simulink library "etherlab_lib"  (Simulink 7.4)
settings: Solver=ode45  SolverMode=SingleTasking  StartTime=0.0  StopTime=10.0  RelTol=1e-3
undefined symbols (not defined in the file or in its folder): Address, baumer_ecatencoder, el320x, el500x, el5101, el5101_0010, EL5151, El5152, el515x, ep41xx, ep43xx, rv, x
(part 2 of 3)

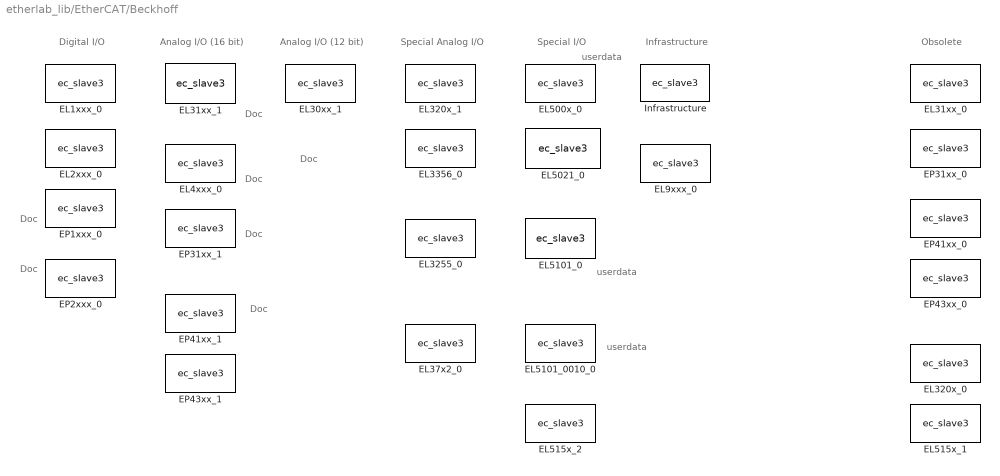
== system etherlab_lib/EtherCAT/Beckhoff ==
  note: Analog I/O (16 bit)
  note: Digital I/O
  note: Analog I/O (12 bit)
  note: Special Analog I/O
  note: Special I/O
  note: Infrastructure
  note: Obsolete
  note: Doc
  note: Doc
  note: Doc
  note: Doc
  note: Doc
  note: Doc
  note: Doc
  note: userdata
  note: userdata
  note: userdata
  EL1xxx_0 : S-Function  FunctionName=ec_slave3  Parameters=Address,rv.SlaveConfig,rv.PortConfig,debug,tsample  SFunctionModules='ecrt_support'  EnableBusSupport=off  mask(EL1xxx){master=0, index=1, model=EL1004, vector=on, tsample=0, debug=0}
      mask prompts: index "Slave Index"; model "Device Model"; vector "Vector Outputs"; tsample "Sample Time"; debug "Debug Level"
      mask help: Beckhoff EtherCAT Digital Input
      mask init:
      | Address = getEtherCATAddress(gcb, master, index, tsample);
      | 
      | rv = el1xxx.configure(model,vector);
      mask Help: web(etherlab_help_path('el1xxx.html'), '-helpbrowser');
      mask StyleString: edit,edit,popup(EL1002|EL1004|EL1004-0010|EL1008|EL1012|EL1014|EL1018|EL1024|EL1034|EL1084|EL1088|EL1094|EL1098|EL1104|EL1114|EL1124|EL1134|EL1144|EL1202|EL1702|EL1712|EL1722|EL1804|EL1808|EL1809|EL1814|EL1819|EL1862|EL1872|EL1889|EL1014-0000-0000),checkbox,edit,edit
      mask Display: fprintf('%s\nM:%i Idx:%s', model, master, mat2str(index))
  EL2xxx_0 : S-Function  FunctionName=ec_slave3  Parameters=Address,rv.SlaveConfig,rv.PortConfig,debug,tsample  SFunctionModules='ecrt_support'  EnableBusSupport=off  mask(EL2xxx){master=0, index=1, model=EL2004, vector=on, diag=on, tsample=-1, debug=0}
      mask prompts: index "Slave Index"; model "Device Model"; vector "Vector Inputs"; diag "Diag Port"; tsample "Sample Time (-1 for inherited)"
      mask help: Beckhoff EtherCAT Digital Output
      mask init:
      | Address = getEtherCATAddress(gcb, master, index, tsample);
      | 
      | rv = el2xxx.configure(model,vector,diag);
      mask Help: web(etherlab_help_path('el2xxx.html'), '-helpbrowser')
      mask StyleString: edit,edit,popup(EL2002|EL2004|EL2008|EL2022|EL2024|EL2032|EL2034|EL2042|EL2084|EL2088|EL2124|EL2202|EL2602|EL2612|EL2622|EL2624|EL2712|EL2722|EL2732|EL2798|EL2808|EL2809|EL2004-0000-0000|EL2032-0000-0000),checkbox,checkbox,edit,edit
      mask CallbackString: ||EtherCATSlaveBlock().setEnable('diag',el2xxx.hasDiag(get_param(gcb,'model')))||||
      mask Display: fprintf('%s\nM:%i Idx:%s', model, master, mat2str(index))
  EL30xx_1 : S-Function  FunctionName=ec_slave3  Parameters=Address,rv.SlaveConfig,rv.PortConfig,debug,tsample  SFunctionModules='ecrt_support'  EnableBusSupport=off  mask(EL30xx){master=0, index=1, model=EL3002, vector=on, status=on, gain=, offset=, tau=, tsample=0, debug=0, filter=Off, opmode=FreeRun, fastop=off}
      mask prompts: index "Slave Index"; model "Device Model"; vector "Vector Output"; status "Status Output"; gain "Output Scale"; offset "Output Offset"; tau "LPF Time Constant (sec)"; tsample "Sample Time"; opmode "Synchronization Mode (1C33:01.0)"; fastop "FastOp Mode (1C33:01.15)"
      mask help: Beckhoff 1,2,4,8-Channel 16-Bit Analog Input
      mask init:
      | Address = getEtherCATAddress(gcb, master, index, tsample);
      | 
      | rv = el30xx_1.configure(model,status,vector,...
      |     EtherCATSlave.configureScale(2^15,gain,offset,tau),...
      |     [filter,opmode,fastop]);
      | 
      | EtherCATSlaveBlock().setPortNames({},...
      |     {rv.PortConfig.output.portname})
      | 
      | set_param(gcb,'AttributesFormatString',...
      |     sprintf('%s %s\nM:%i Idx:%s',...
      |             model,rv.function,master,mat2str(index)))
      settings: AttributesFormatString=|
      | EL3002 +-10V
      | M:0 Idx:1
      mask StyleString: edit,edit,popup(EL3001|EL3002|EL3004|EL3008|EL3011|EL3012|EL3014|EL3021|EL3022|EL3024|EL3041|EL3042|EL3044|EL3048|EL3051|EL3052|EL3054|EL3058|EL3061|EL3062|EL3062-0030|EL3064|EL3068),checkbox,checkbox,edit,edit,edit,edit,edit,popup(Off|50Hz FIR|60Hz FIR|IIR 1|IIR 2|IIR 3|IIR 4|IIR 5|IIR 6|IIR 7|IIR 8),popup(FreeRun|FrameTriggered SM2),checkbox
      mask CallbackString:
      | ||||||||||EtherCATSlaveBlock().setEnable({'opmode','fastop'},...
      |         strcmp(get_param(gcb,'filter'),'Off'));
      | ||
      mask TabNameString: Main,Main,Main,Main,Main,Main,Main,Main,Main,Main,Filter,Filter,Filter
      mask Display:
      | port_label('output', 1, 'Value')
      | port_label('output', 2, 'Status')
  EL31xx_0 : S-Function  LoadFcn=|  FunctionName=ec_slave3  Parameters=Address,rv.SlaveConfig,rv.PortConfig,debug,tsample  SFunctionModules='ecrt_support'  EnableBusSupport=off  mask(EL31xx){master=0, index=1, model=EL3102, dc=DC-Synchron, vector=on, raw=off, scale=, offset=, tau=, tsample=0, debug=0}
      | el31xx('check')                              
      | if ~strcmp(bdroot(gcb),'etherlab_lib')       
      |    disp([gcb ' is obsolete. Please replace'])
      | end
      mask prompts: index "Slave Index"; model "Device Model"; dc "Distributed Clock"; vector "Vector Output"; raw "Raw output"; scale "Output Scale"; offset "Output Offset"; tau "LPF Time Constant (sec)"; tsample "Sample Time"
      mask help:
      | Beckhoff 2,4,8-Channel 16-Bit Analog Input with Distributed Clocks
      |
      | Status output is not supported
      mask init:
      | masterStr = '';
      | positionStr = '';
      | [Address masterStr positionStr] = ...
      |     getEtherCATAddress(gcb, master, index, tsample);
      | 
      | el31xx('set');  % Report errors
      | 
      | rv = get_param(gcb,'UserData');
      mask Help:
      | This block generically implements the EtherCAT 16-Bit Analog Input Terminal for various models.
      | <p/>
      | The following Terminals are supported:
      | <center>
      | <table width="80%">
      | <tr><td>EL3102,4,8</td><td>-10..10V Voltage Input</td></tr>
      | <tr><td>EL3112,4   </td><td>0..20mA Current Input</td></tr>
      | <tr><td>EL3122,4   </td><td>4..20mA Current Input</td></tr>
      | <tr><td>EL3142,4,8</td><td>0..20mA Current Input</td></tr>
      | <tr><td>EL3152,4,8</td><td>4..20mA Current Input</td></tr>
      | <tr><td>EL3162,4,8</td><td>0..10V Voltage Input</td></tr>
      | </table>
      | </center>
      | <p/>
      | Choose and set the following options:
      | <h4>Master:</h4>
      | Set the EtherCAT Master of this terminal.
      | 
      | <h4>Slave Index:</h4>
      | Set the EtherCAT slave index. Following address formats are allowed:
      | <ol>
      | <li> Absolute addressing: a scalar number <<b><tt>n</tt></b>> representing the (zero based) absolute position in the bus.
      | <li> SSId addressing: the Secondary Slave (or 'Alias') Addressing has the form <<b><tt>[alias position]</tt></b>> where <b><tt>alias</tt></b> is the Secondary Slave Id of the EtherCAT slave and <b><tt>position</tt></b> is the offset after the slave with the given <b><tt>alias</tt></b>. The SSId has to be preprogrammed into the slave with other service tools (see 'ethercat alias --help').
      | </ol>
      | 
      | <h4>Device Model:</h4>
      | Choose the model at the Indexed position of the master.
      | 
      | <h4>Output Type:</h4>
      | <ul>
      | <li>Choose <b>Vector Output</b> to have a single output as a vector
      | with a size corresponding to the channel count of the terminal. This mode also allows a status output port to be displayed. <br/>
      | <li>Choose <b>Separate Outputs</b> to have one output for every channel.
      | </ul>
      | <h4>Output Full Scale</h4>
      | When <b>Output Data Type</b> is set to <b>Double with scale and offset</b>, the block's output value at full scale terminal input can be set here.
      | 
      | <h4>Output Offset</h4>
      | When <b>Output Data Type</b> is set to <b>Double with scale and offset</b>, the blocks output at zero terminal input can be set here. Note that the Full Scale above is also increased by this amount. Note furthermore that this corresponds to the minimum input for terminals such as 4..20mA.
      | 
      | <h4>Output Data Type</h4>
      | Choose the block's output data type for the output signal. Available are:
      | <ul>
      | <li><b><tt>Raw</tt></b> outputting the internal raw value as <tt>int16_T</tt> or <tt>uint16_T</tt> as appropriate
      | <li><b><tt>Double</tt></b> outputting 0..10, -10..10, 0..0.02 and 0.004..0.02 depending on the Model as appropriate
      | <li><b><tt>Double with scale and offset</tt></b>, allowing the output to be scaled with an offset.
      | </ul>
      | 
      | <p>
      | Choosing <b>Status Output</b> provides a port of type <tt>uint8_T</tt> where the status is presented. This is only enabled when <b>Vector Output</b> is selected. Terminal input over- and underrange can be detected using this output. See the terminal's documentation.
      | 
      | <h4>Output Filter</h4>
      | When not in <b>Raw</b> mode, the <b>Output Filter</b> checkbox becomes available, allowing the use of an internal low pass filter. Enter the <b>LPF Time Constant</b> for the filter in the field below.
      | <br>For continuous sample time systems (0 in Sample Time), the filter is also continuous. Discrete samples systems (Sample Time > 0) uses an equivalent discrete low pass filter with a similar time constant.
      | 
      | <p>
      | Set the <b>Sample Time</b> for the block. <tt>0</tt> is continuous sample time (runs at the model's base rate). Setting <tt>-1</tt> will try to set the time using back propagation.
      mask StyleString: edit,edit,popup(EL3101|EL3102|EL3104|EL3111|EL3112|EL3114|EL3121|EL3122|EL3124|EL3141|EL3142|EL3142-010|EL3144|EL3151|EL3152|EL3154|EL3161|EL3162|EL3164),popup(Free Run|DC-Synchron|DC-Synchron (input based)),checkbox,checkbox,edit,edit,edit,edit,edit
      mask CallbackString: ||el31xx('set')|el31xx('set')|el31xx('set')||||||
      mask Display:
      | fprintf('%s\n%s AIn\nM:%s Idx:%s', ...
      |     model, rv.SlaveConfig.function, masterStr, positionStr)
  EL31xx_1 : S-Function  FunctionName=ec_slave3  Parameters=Address,rv.SlaveConfig,rv.PortConfig,debug,tsample  SFunctionModules='ecrt_support'  EnableBusSupport=off  mask(EL31xx){master=0, index=1, model=EL3102, vector=on, status=on, filter=Off, gain=, offset=, tau=, tsample=0, debug=, dc_mode=Free Run/SM-Synchron, dc_assign_activate=, dc_cycle0=[], dc_cycle0_factor=[], dc_shift0=[], dc_shift0_factor=[], dc_shift0_input=off, dc_cycle1=[], dc_cycle1_factor=[], dc_shift1=[], dc_shift1_factor=[]}
      mask prompts: index "Slave Index"; model "Device Model"; vector "Vector Output"; status "Status output"; gain "Output Gain"; offset "Output Offset"; tau "LPF Time Constant (sec)"; tsample "Sample Time"; dc_mode "Mode"; dc_assign_activate "Assign Activate"; dc_cycle0 "Cycle Time Sync 0"; dc_cycle0_factor "Factor"; dc_shift0 "Shift Time Sync0"; dc_shift0_factor "Factor"; dc_shift0_input "Shift Time0 Input"; dc_cycle1 "Cycle Time Sync1"; dc_cycle1_factor "Factor"; dc_shift1 "Shift Time Sync1"; dc_shift1_factor "Factor"
      mask help: Beckhoff 2,4,8-Channel 16-Bit Analog Input with Distributed Clocks
      mask init:
      | Address = getEtherCATAddress(gcb, master, index, tsample);
      | 
      | rv = el31xx_1.configure(model,status,vector,...
      |     EtherCATSlave.configureScale(2^15,gain,offset,tau),...
      |     [dc_mode, dc_assign_activate, ...
      |      dc_cycle0, dc_cycle0_factor, ...
      |      dc_shift0, dc_shift0_factor, dc_shift0_input, ...
      |      dc_cycle1, dc_cycle1_factor, ...
      |      dc_shift1, dc_shift1_factor], ...
      |      filter);
      |  
      | EtherCATSlaveBlock().setPortNames({},...
      |     {rv.PortConfig.output.portname})
      | 
      | set_param(gcb,'AttributesFormatString',...
      |     sprintf('%s %s\nM:%i Idx:%s',...
      |             model,rv.function,master,mat2str(index)))
      settings: AttributesFormatString=|
      | EL3102 +-10V
      | M:0 Idx:1
      mask Help:
      | This block generically implements the EtherCAT 16-Bit Analog Input Terminal for various models.
      | <p/>
      | The following Terminals are supported:
      | <center>
      | <table width="80%">
      | <tr><td>EL3102,4,8</td><td>-10..10V Voltage Input</td></tr>
      | <tr><td>EL3112,4   </td><td>0..20mA Current Input</td></tr>
      | <tr><td>EL3122,4   </td><td>4..20mA Current Input</td></tr>
      | <tr><td>EL3142,4,8</td><td>0..20mA Current Input</td></tr>
      | <tr><td>EL3152,4,8</td><td>4..20mA Current Input</td></tr>
      | <tr><td>EL3162,4,8</td><td>0..10V Voltage Input</td></tr>
      | </table>
      | </center>
      | <p/>
      | Choose and set the following options:
      | <h4>Master:</h4>
      | Set the EtherCAT Master of this terminal.
      | 
      | <h4>Slave Index:</h4>
      | Set the EtherCAT slave index. Following address formats are allowed:
      | <ol>
      | <li> Absolute addressing: a scalar number <<b><tt>n</tt></b>> representing the (zero based) absolute position in the bus.
      | <li> SSId addressing: the Secondary Slave (or 'Alias') Addressing has the form <<b><tt>[alias position]</tt></b>> where <b><tt>alias</tt></b> is the Secondary Slave Id of the EtherCAT slave and <b><tt>position</tt></b> is the offset after the slave with the given <b><tt>alias</tt></b>. The SSId has to be preprogrammed into the slave with other service tools (see 'ethercat alias --help').
      | </ol>
      | 
      | <h4>Device Model:</h4>
      | Choose the model at the Indexed position of the master.
      | 
      | <h4>Output Type:</h4>
      | <ul>
      | <li>Choose <b>Vector Output</b> to have a single output as a vector
      | with a size corresponding to the channel count of the terminal. This mode also allows a status output port to be displayed. <br/>
      | <li>Choose <b>Separate Outputs</b> to have one output for every channel.
      | </ul>
      | <h4>Output Full Scale</h4>
      | When <b>Output Data Type</b> is set to <b>Double with scale and offset</b>, the block's output value at full scale terminal input can be set here.
      | 
      | <h4>Output Offset</h4>
      | When <b>Output Data Type</b> is set to <b>Double with scale and offset</b>, the blocks output at zero terminal input can be set here. Note that the Full Scale above is also increased by this amount. Note furthermore that this corresponds to the minimum input for terminals such as 4..20mA.
      | 
      | <h4>Output Data Type</h4>
      | Choose the block's output data type for the output signal. Available are:
      | <ul>
      | <li><b><tt>Raw</tt></b> outputting the internal raw value as <tt>int16_T</tt> or <tt>uint16_T</tt> as appropriate
      | <li><b><tt>Double</tt></b> outputting 0..10, -10..10, 0..0.02 and 0.004..0.02 depending on the Model as appropriate
      | <li><b><tt>Double with scale and offset</tt></b>, allowing the output to be scaled with an offset.
      | </ul>
      | 
      | <p>
      | Choosing <b>Status Output</b> provides a port of type <tt>uint8_T</tt> where the status is presented. This is only enabled when <b>Vector Output</b> is selected. Terminal input over- and underrange can be detected using this output. See the terminal's documentation.
      | 
      | <h4>Output Filter</h4>
      | When not in <b>Raw</b> mode, the <b>Output Filter</b> checkbox becomes available, allowing the use of an internal low pass filter. Enter the <b>LPF Time Constant</b> for the filter in the field below.
      | <br>For continuous sample time systems (0 in Sample Time), the filter is also continuous. Discrete samples systems (Sample Time > 0) uses an equivalent discrete low pass filter with a similar time constant.
      | 
      | <p>
      | Set the <b>Sample Time</b> for the block. <tt>0</tt> is continuous sample time (runs at the model's base rate). Setting <tt>-1</tt> will try to set the time using back propagation.
      mask StyleString: edit,edit,popup(EL3101|EL3102|EL3104|EL3111|EL3112|EL3114|EL3121|EL3122|EL3124|EL3141|EL3142|EL3142-0010|EL3144|EL3151|EL3152|EL3154|EL3161|EL3162|EL3164),checkbox,checkbox,popup(Off|50Hz FIR|60Hz FIR|IIR 1|IIR 2|IIR 3|IIR 4|IIR 5|IIR 6|IIR 7|IIR 8),edit,edit,edit,edit,edit,popup(Free Run/SM-Synchron|DC-Synchron|DC-Synchron (input based)|Custom),edit,min,max,min,max,checkbox,min,max,min,max
      mask CallbackString: |||||||||||EtherCATSlaveBlock().updateCustomDCEnable()||||||||||
      mask TabNameString: Main,Main,Main,Main,Main,Main,Main,Main,Main,Main,Main,Distributed Clocks,Distributed Clocks,Distributed Clocks,Distributed Clocks,Distributed Clocks,Distributed Clocks,Distributed Clocks,Distributed Clocks,Distributed Clocks,Distributed Clocks,Distributed Clocks
      mask Display:
      | port_label('output', 1, 'Value')
      | port_label('output', 2, 'Status')
  EL320x_0 : S-Function  LoadFcn=el320x('check')  FunctionName=ec_slave3  Parameters=Address,rv.SlaveConfig,rv.PortConfig,debug,tsample  SFunctionModules='ecrt_support'  EnableBusSupport=off  mask(EL320x){master=0, index=1, model=EL3204, rtd=0, technology=2, filter=50 Hz, vector=on, enable_status=on, tsample=0, debug=0}
      mask prompts: index "Slave Index"; model "Device Model"; rtd "RTD-Element (CoE 80x0:19)"; technology "Connection Technology (CoE 80x0:1A)"; filter "Filter (CoE 8000:15)"; vector "Vector Output"; enable_status "Status Port"; tsample "Sample Time"
      mask help: Beckhoff 1, 2, 4-Channel Input Terminal Pt100 (RTD)
      mask init:
      | masterStr = '';
      | positionStr = '';
      | [Address masterStr positionStr] = ...
      |     getEtherCATAddress(gcb,master,index,tsample);
      | SdoConfig = [];
      | 
      | rv = get_param(gcbh,'UserData');
      | 
      | count = numel(rv.SlaveConfig.sm{1}{3});
      | 
      | err = {};
      | if numel(rtd) == 1
      |     rtd = repmat(rtd,1,count);
      | elseif numel(rtd) ~= count
      |     err = {['- Mask option "RTD Element"' ...
      |         ' is not a scalar or vector with ' ...
      |         num2str(count) ' elements']};
      | end
      | 
      | if numel(technology) == 1
      |     technology = repmat(technology,1,count);
      | elseif numel(technology) ~= count
      |     err = horzcat(err, ['- Mask option "Connection Technology"' ...
      |         ' is not a scalar or vector with ' ...
      |         num2str(count) ' elements']);
      | end
      | 
      | if ~isempty(err)
      |     errordlg(err,gcb);
      |     return
      | end
      | 
      | rv.SlaveConfig.sdo = num2cell(vertcat(...
      |     [hex2dec('8000'),6,8,1],...
      |     [hex2dec('8000'),hex2dec('15'),16,filter+1],...
      |     horzcat(repmat(hex2dec('8000') + 16*(0:count-1)',2,1),...
      |             [hex2dec('19')*ones(count,1);hex2dec('1a')*ones(count,1)],...
      |             16*ones(count*2,1),...
      |             vertcat(reshape(rtd,[],1),...
      |                     reshape(technology,[],1)))));
      mask Help: web(etherlab_help_path('el320x.html'), '-helpbrowser');
      mask StyleString: edit,edit,popup(EL3201|EL3201-0010|EL3201-0020|EL3202|EL3202-0010|EL3204),edit,edit,popup(50 Hz|60 Hz|100 Hz|500 Hz|1 kHz|2 kHz|3.75 kHz|7.5 kHz|15 kHz|30 kHz|5 Hz|10 Hz),checkbox,checkbox,edit,edit
      mask CallbackString: ||el320x('set');||||el320x('set');|el320x('set');||
      mask Display: fprintf('%s\nRTD In\n%i Idx:%s', model, master, mat2str(index))
  EL320x_1 : S-Function  FunctionName=ec_slave3  Parameters=Address,rv.SlaveConfig,rv.PortConfig,debug,tsample  SFunctionModules='ecrt_support'  EnableBusSupport=off  mask(EL320x){master=0, index=1, model=EL3204, filter=Off, vector=on, status=on, tsample=0, debug=, rtd1=Pt100 -200...850C, technology1=2-wire, calib1=0, rtd2=Pt100 -200...850C, technology2=2-wire, calib2=0, rtd3=Pt100 -200...850C, technology3=2-wire, calib3=0, rtd4=Pt100 -200...850C, technology4=2-wire, calib4=0}
      mask prompts: index "Slave Index"; model "Device Model"; vector "Vector Output"; status "Status Port"; tsample "Sample Time"; rtd1 "RTD-Element"; technology1 "Technology"; calib1 "Wire Calibration (1/32 Ohm)"; rtd2 "RTD-Element"; technology2 "Technology"; calib2 "Wire Calibration (1/32 Ohm)"; rtd3 "RTD-Element"; technology3 "Technology"; calib3 "Wire Calibration (1/32 Ohm)"; rtd4 "RTD-Element"; technology4 "Technology"; calib4 "Wire Calibration (1/32 Ohm)"
      mask help: Beckhoff 1, 2, 4-Channel Input Terminal Pt100 (RTD)
      mask init:
      | Address = getEtherCATAddress(gcb,master,index,tsample);
      | 
      | % rv.SlaveConfig.sdo = num2cell(vertcat(...
      | %     [hex2dec('8000'),6,8,1],...
      | %     [hex2dec('8000'),hex2dec('15'),16,filter+1],...
      | %     horzcat(repmat(hex2dec('8000') + 16*(0:count-1)',2,1),...
      | %             [hex2dec('19')*ones(count,1);hex2dec('1a')*ones(count,1)],...
      | %             16*ones(count*2,1),...
      | %             vertcat(reshape(rtd,[],1),...
      | %                     reshape(technology,[],1)))));
      | % rv.PortConfig = [];
      | % rv.SlaveConfig = [];
      | 
      | rv = el320x_1.configure(model,status,vector,filter,...
      |     [rtd1,rtd2,rtd3,rtd4],...
      |     [technology1,technology2,technology3,technology4],...
      |     [calib1,calib2,calib3,calib4]);
      mask Help: web(etherlab_help_path('el320x.html'), '-helpbrowser');
      mask StyleString: edit,edit,popup(EL3201|EL3201-0010|EL3201-0020|EL3202|EL3202-0010|EL3204),popup(Off|50 Hz|60 Hz|100 Hz|500 Hz|1 kHz|2 kHz|3.75 kHz|7.5 kHz|15 kHz|30 kHz|5 Hz|10 Hz),checkbox,checkbox,edit,edit,popup(Pt100 -200...850C|Ni100 -60...250C|Pt1000 -200...850C|Pt500 -200...850C|Pt200 -200...850C|Ni1000 -60...250C|Ni1000 100C: 1500 Ohm (-30...60C)|Ni120 -60...320C|1/16 Ohm (10 .. 4095 Ohm) |1/64 Ohm (10 .. 1047 Ohm) |KT100/110/130/210/230 KTY10/11/13/16/19  |KTY81/82-110/120/150 (-50...150C)|KTY81-121|KTY81-122|KTY81-151|KTY81-152|KTY81/82-210/220/250|KTY81-221|KTY81-222|KTY81-251|KTY81-252|KTY83-110/120/150 (-50...175C)|KTY83-121|KTY83-122|KTY83-151|KTY83-152|KTY84-130/150 (-40...300C)|KTY84-151|KTY21/23-6 (-50...150C)|KTY1x-5|KTY1x-7|KTY21/23-5|KTY21/23-7),popup(2-wire|3-wire|4-wire|Not connected),edit,popup(Pt100 -200...850C|Ni100 -60...250C|Pt1000 -200...850C|Pt500 -200...850C|Pt200 -200...850C|Ni1000 -60...250C|Ni1000 100C: 1500 Ohm (-30...60C)|Ni120 -60...320C|1/16 Ohm (10 .. 4095 Ohm) |1/64 Ohm (10 .. 1047 Ohm) |KT100/110/130/210/230 KTY10/11/13/16/19  |KTY81/82-110/120/150 (-50...150C)|KTY81-121|KTY81-122|KTY81-151|KTY81-152|KTY81/82-210/220/250|KTY81-221|KTY81-222|KTY81-251|KTY81-252|KTY83-110/120/150 (-50...175C)|KTY83-121|KTY83-122|KTY83-151|KTY83-152|KTY84-130/150 (-40...300C)|KTY84-151|KTY21/23-6 (-50...150C)|KTY1x-5|KTY1x-7|KTY21/23-5|KTY21/23-7),popup(2-wire|3-wire|4-wire|Not connected),edit,popup(Pt100 -200...850C|Ni100 -60...250C|Pt1000 -200...850C|Pt500 -200...850C|Pt200 -200...850C|Ni1000 -60...250C|Ni1000 100C: 1500 Ohm (-30...60C)|Ni120 -60...320C|1/16 Ohm (10 .. 4095 Ohm) |1/64 Ohm (10 .. 1047 Ohm) |KT100/110/130/210/230 KTY10/11/13/16/19  |KTY81/82-110/120/150 (-50...150C)|KTY81-121|KTY81-122|KTY81-151|KTY81-152|KTY81/82-210/220/250|KTY81-221|KTY81-222|KTY81-251|KTY81-252|KTY83-110/120/150 (-50...175C)|KTY83-121|KTY83-122|KTY83-151|KTY83-152|KTY84-130/150 (-40...300C)|KTY84-151|KTY21/23-6 (-50...150C)|KTY1x-5|KTY1x-7|KTY21/23-5|KTY21/23-7),popup(2-wire|3-wire|4-wire|Not connected),edit,popup(Pt100 -200...850C|Ni100 -60...250C|Pt1000 -200...850C|Pt500 -200...850C|Pt200 -200...850C|Ni1000 -60...250C|Ni1000 100C: 1500 Ohm (-30...60C)|Ni120 -60...320C|1/16 Ohm (10 .. 4095 Ohm) |1/64 Ohm (10 .. 1047 Ohm) |KT100/110/130/210/230 KTY10/11/13/16/19  |KTY81/82-110/120/150 (-50...150C)|KTY81-121|KTY81-122|KTY81-151|KTY81-152|KTY81/82-210/220/250|KTY81-221|KTY81-222|KTY81-251|KTY81-252|KTY83-110/120/150 (-50...175C)|KTY83-121|KTY83-122|KTY83-151|KTY83-152|KTY84-130/150 (-40...300C)|KTY84-151|KTY21/23-6 (-50...150C)|KTY1x-5|KTY1x-7|KTY21/23-5|KTY21/23-7),popup(2-wire|3-wire|4-wire|Not connected),edit
      mask TabNameString: Main,Main,Main,Main,Main,Main,Main,Main,Sensor 1,Sensor 1,Sensor 1,Sensor 2,Sensor 2,Sensor 2,Sensor 3,Sensor 3,Sensor 3,Sensor 4,Sensor 4,Sensor 4
      mask Display: fprintf('%s\nRTD In\n%i Idx:%s', model, master, mat2str(index))
  EL3255_0 : S-Function  FunctionName=ec_slave3  Parameters=Address,rv.SlaveConfig,rv.PortConfig,debug,tsample  SFunctionModules='ecrt_support'  EnableBusSupport=off  mask(EL3255){master=0, index=1, model=EL3255, channels=1, vector=on, gain=[], offset=[], filter=[], tsample=0, debug=0, dc_mode=Free Run/SM-Synchron, dc_assign_activate=hex2dec('700'), dc_cycle0=[], dc_cycle0_factor=[], dc_shift0=0, dc_shift0_factor=0, dc_shift0_input=off, dc_cycle1=[], dc_cycle1_factor=[], dc_shift1=20000, dc_shift1_factor=0, x8000_06=off, x8000_15=50 Hz, x8000_1c=Off (up to 10 kOhm), x8010_1c=Off (up to 10 kOhm), x8020_1c=Off (up to 10 kOhm), x8030_1c=Off (up to 10 kOhm), x8040_1c=Off (up to 10 kOhm)}
      mask prompts: index "Slave Index"; model "Device Model"; channels "Active Channels"; vector "Vector Outputs"; filter "Filter time"; tsample "Sample Time"; debug "Debug Level"; dc_mode "Distributed Clock"; dc_assign_activate "Assign Activate"; dc_cycle0 "Cycle Time Sync 0"; dc_cycle0_factor "Factor"; dc_shift0 "Shift Time Sync0"; dc_shift0_factor "Factor"; dc_shift0_input "Shift Time0 Input"; dc_cycle1 "Cycle Time Sync1"; dc_cycle1_factor "Factor"; dc_shift1 "Shift Time Sync1"; dc_shift1_factor "Factor"; x8000_06 "Enable Filter (#x8000:06)"; x8000_15 "Filter settings (#x8000:15)"; x8000_1c "Load resistance 1"; x8010_1c "Load resistance 2"; x8020_1c "Load resistance 3"; x8030_1c "Load resistance 4"; x8040_1c "Load resistance 5"
      mask help: Beckhoff EtherCAT 5Ch. potentiometer measurement with sensor supply
      mask init:
      | Address = getEtherCATAddress(gcb, master, index, tsample);
      | 
      | rv = el3255.configure(model,channels,vector,...
      |     [dc_mode, dc_assign_activate, ...
      |     dc_cycle0, dc_cycle0_factor,...
      |     dc_shift0, dc_shift0_factor, dc_shift0_input,...
      |     dc_cycle1, dc_cycle1_factor,...
      |     dc_shift1, dc_shift1_factor], ...
      |     EtherCATSlave.configureScale(2^15,gain,offset,filter),...
      |     [x8000_06, x8000_15, ...
      |      x8000_1c, x8010_1c, x8020_1c, x8030_1c, x8040_1c]);
      |  
      | EtherCATSlaveBlock().setPortNames(...
      |     {}, {rv.PortConfig.output.portname});
      | 
      | set_param(gcb,'AttributesFormatString',...
      |     sprintf('%s\nM:%i Idx:%s',...
      |             model,master,mat2str(index)))
      settings: AttributesFormatString=|
      | EL3255
      | M:0 Idx:1
      mask Help: web(etherlab_help_path('el3255.html'), '-helpbrowser');
      mask StyleString: edit,edit,popup(EL3255),popup(1|1..2|1..3|1..4|1..5),checkbox,edit,edit,edit,edit,edit,popup(Free Run/SM-Synchron|DC-Synchron|DC-Synchron (input based)|Custom),edit,min,max,min,max,checkbox,min,max,min,max,checkbox,popup(50 Hz|60 Hz|100 Hz|500 Hz|1 kHz|2 kHz|3.75 kHz|7.5 kHz|15 kHz|30 kHz|5 Hz|10 Hz),popup(Off (up to 10 kOhm)|25 kOhm|50 kOhm),popup(Off (up to 10 kOhm)|25 kOhm|50 kOhm),popup(Off (up to 10 kOhm)|25 kOhm|50 kOhm),popup(Off (up to 10 kOhm)|25 kOhm|50 kOhm),popup(Off (up to 10 kOhm)|25 kOhm|50 kOhm)
      mask CallbackString: ||||||||||EtherCATSlaveBlock(gcbh).updateCustomDCEnable();|||||||||||||||||
      mask TabNameString: Main,Main,Main,Main,Main,Main,Main,Main,Main,Main,Distributed Clocks,Distributed Clocks,Distributed Clocks,Distributed Clocks,Distributed Clocks,Distributed Clocks,Distributed Clocks,Distributed Clocks,Distributed Clocks,Distributed Clocks,Distributed Clocks,CoE,CoE,CoE,CoE,CoE,CoE,CoE
      mask Display: port_label('output', 1, 'Ch. 1')
  EL3356_0 : S-Function  FunctionName=ec_slave3  Parameters=Address,rv.SlaveConfig,rv.PortConfig,debug,tsample  SFunctionModules='ecrt_support'  EnableBusSupport=off  mask(EL3356){master=0, index=1, model=EL3356-0010, adc=off, scale=, offset=, tau=, tsample=0, debug=0, dc_mode=SM-Synchron, dc_assign_activate=hex2dec('320'), dc_cycle0=[], dc_cycle0_factor=[], dc_shift0=0, dc_shift0_factor=0, dc_shift0_input=off, dc_cycle1=[], dc_cycle1_factor=[], dc_shift1=0, dc_shift1_factor=0, x8000_01=off, x8000_02=off, x8000_03=on, x8000_04=on, x8000_05=on, x8000_11=FIR 50 Hz, x8000_12=FIR 50 Hz, x8000_13=10, x8000_14=hex2dec(num2hex(single(20))), x8000_29=1000, x8000_2A=5, x8000_31=1800, x8000_32=10, x8010_06=off, x8010_15=50 Hz FIR, x8020_06=off, x8020_15=50 Hz FIR}
      mask prompts: index "Slave Index"; model "Device Model"; adc "2 ch ADC only"; scale "Output Scale"; offset "Output Offset"; tau "LPF Time Constant (sec)"; tsample "Sample Time"; dc_mode "Mode"; dc_assign_activate "Assign Activate"; dc_cycle0 "Cycle Time Sync 0"; dc_cycle0_factor "Factor"; dc_shift0 "Shift Time Sync0"; dc_shift0_factor "Factor"; dc_shift0_input "Shift Time0 Input"; dc_cycle1 "Cycle Time Sync1"; dc_cycle1_factor "Factor"; dc_shift1 "Shift Time Sync1"; dc_shift1_factor "Factor"; x8000_01 "Mode 0 Enable Filter (#x8000:01)"; x8000_02 "Mode 1 Enable Filter (#x8000:02)"; x8000_03 "Mode 0 Enable Averager (#x8000:03)"; x8000_04 "Mode 1 Enable Averager (#x8000:04)"; x8000_05 "Symmetric Reference Potential (#x8000:05)"; x8000_11 "Mode 0 Filter (#x8000:11)"; x8000_12 "Mode 1 Filter (#x8000:12)"; x8000_13 "Dynamic filter change time [0.01s] (#x8000:13)"; x8000_14 "Dynamic filter delta (#x8000:14) (binary value)"; x8000_29 "Steady state window (#x8000:29)"; x8000_2A "Steady state tolerance (#x8000:2a)"; x8000_31 "Calibration interval [100ms] (#x8000:31)"; x8000_32 "Test interval (#x8000:32)"; x8010_06 "Enable ch. 1 filter (#x8010:06)"; x8010_15 "Ch.1 filter settings (#x8010:15)"; x8020_06 "Enable ch.2 filter (#x8020:06)"; x8020_15 "Ch.2 filter settings (#x8020:15)"
      mask help: Beckhoff DMS Input with Distributed Clocks
      mask init:
      | Address = getEtherCATAddress(gcb, master, index, tsample);
      | 
      | rv = el3356.configure(model,adc,...
      |     [dc_mode, dc_assign_activate, ...
      |     dc_cycle0, dc_cycle0_factor,...
      |     dc_shift0, dc_shift0_factor, dc_shift0_input,...
      |     dc_cycle1, dc_cycle1_factor,...
      |     dc_shift1, dc_shift1_factor], ...
      |     EtherCATSlave.configureScale(2^31,scale,offset,tau),...
      |     [x8000_01, x8000_02, x8000_03, x8000_04, x8000_05, ...
      |      x8000_11, x8000_12, x8000_13, x8000_14, x8000_29, ...
      |      x8000_2A, x8000_31, x8000_32, ...
      |      x8010_06, x8010_15, ...
      |      x8020_06, x8020_15]);
      |  
      | EtherCATSlaveBlock().setPortNames(...
      |     {rv.PortConfig.input.portname},...
      |     {rv.PortConfig.output.portname});
      | 
      | set_param(gcb,'AttributesFormatString',...
      |     sprintf('%s\nM:%i Idx:%s',...
      |             model,master,mat2str(index)))
      settings: AttributesFormatString=|
      | EL3356-0010
      | M:0 Idx:1
      mask Help: web(etherlab_help_path('el3356.html'), '-helpbrowser');
      mask StyleString: edit,edit,popup(EL3356|EL3356-0010),checkbox,edit,edit,edit,edit,edit,popup(SM-Synchron|DC-Synchron|DC-Synchron (input based)|Custom),edit,min,max,min,max,checkbox,min,max,min,max,checkbox,checkbox,checkbox,checkbox,checkbox,popup(FIR 50 Hz|FIR 60 Hz|IIR 1|IIR 2|IIR 3|IIR 4|IIR 5|IIR 6|IIR 7|IIR 8|Dynamic IIR),popup(FIR 50 Hz|FIR 60 Hz|IIR 1|IIR 2|IIR 3|IIR 4|IIR 5|IIR 6|IIR 7|IIR 8|Dynamic IIR),edit,edit,edit,edit,edit,edit,checkbox,popup(50 Hz FIR|60 Hz FIR|IIR 1|IIR 2|IIR 3|IIR 4|IIR 5|IIR 6|IIR 7|IIR 8),checkbox,popup(50 Hz FIR|60 Hz FIR|IIR 1|IIR 2|IIR 3|IIR 4|IIR 5|IIR 6|IIR 7|IIR 8)
      mask CallbackString:
      | ||b = EtherCATSlaveBlock(gcb);
      | model = get_param(gcbh,'model');
      | b.updateDCVisibility(~isempty(el3356.getDC(model)));
      | b.updateSDOVisibility(el3356.getSDO(model));
      | |||||||EtherCATSlaveBlock(gcbh).updateCustomDCEnable();|||||||||||||||||||||||||||
      mask TabNameString: Main,Main,Main,Main,Main,Main,Main,Main,Main,Distributed Clocks,Distributed Clocks,Distributed Clocks,Distributed Clocks,Distributed Clocks,Distributed Clocks,Distributed Clocks,Distributed Clocks,Distributed Clocks,Distributed Clocks,Distributed Clocks,CoE #x8000,CoE #x8000,CoE #x8000,CoE #x8000,CoE #x8000,CoE #x8000,CoE #x8000,CoE #x8000,CoE #x8000,CoE #x8000,CoE #x8000,CoE #x8000,CoE #x8000,CoE #x80x0,CoE #x80x0,CoE #x80x0,CoE #x80x0
      mask Display:
      | port_label('input', 1, 'Ctrl')
      | port_label('output', 1, 'RMB')
      | port_label('output', 2, 'Status')
  EL37x2_0 : S-Function  FunctionName=ec_slave3  Parameters=Address,rv.SlaveConfig,rv.PortConfig,debug,tsample  SFunctionModules='ecrt_support'  EnableBusSupport=off  mask(EL37x2){master=0, index=1, model=EL3702, one_ch=off, scale=, offset=, tsample=0, debug=0, dc_mode=10, dc_assign_activate=hex2dec('730'), dc_cycle0=0, dc_cycle0_factor=-10     % 10-times OS, dc_shift0=-10000, dc_shift0_factor=1, dc_shift0_input=off, dc_cycle1=0, dc_cycle1_factor=-1, dc_shift1=0, dc_shift1_factor=0}
      mask prompts: index "Slave Index"; model "Device Model"; one_ch "1 Ch. only"; scale "Output Scale"; offset "Output Offset"; tsample "Sample Time"; dc_mode "Mode/Oversampling"; dc_assign_activate "Assign Activate"; dc_cycle0 "Cycle Time Sync 0 [ns]"; dc_cycle0_factor "Factor"; dc_shift0 "Shift Time Sync0 [ns]"; dc_shift0_factor "Factor"; dc_shift0_input "Shift Time0 Input"; dc_cycle1 "Cycle Time Sync1 [ns]"; dc_cycle1_factor "Factor"; dc_shift1 "Shift Time Sync1 [ns]"; dc_shift1_factor "Factor"
      mask help: Beckhoff oversampling analog input
      mask init:
      | Address = getEtherCATAddress(gcb, master, index, tsample);
      | 
      | rv = el37x2.configure(model,one_ch,...
      |     [dc_mode, dc_assign_activate, ...
      |     dc_cycle0, dc_cycle0_factor,...
      |     dc_shift0, dc_shift0_factor, dc_shift0_input,...
      |     dc_cycle1, dc_cycle1_factor,...
      |     dc_shift1, dc_shift1_factor], ...
      |     EtherCATSlave.configureScale(2^15,scale,offset));
      |  
      | EtherCATSlaveBlock().setPortNames(...
      |     {},...
      |     {rv.PortConfig.output.portname});
      settings: AttributesFormatString=%<model>\nM:%<master> Idx:%<index>
      mask Help: web(etherlab_help_path('el37x2.html'), '-helpbrowser');
      mask StyleString: edit,edit,popup(EL3702|EL3742),checkbox,edit,edit,edit,edit,popup(1|2|3|4|5|8|10|16|20|25|32|40|50|100|Custom),edit,min,max,min,max,checkbox,min,max,min,max
      mask CallbackString: ||||||||EtherCATSlaveBlock(gcbh).updateCustomDCEnable();||||||||||
      mask TabNameString: Main,Main,Main,Main,Main,Main,Main,Main,Oversampling/DC,Oversampling/DC,Oversampling/DC,Oversampling/DC,Oversampling/DC,Oversampling/DC,Oversampling/DC,Oversampling/DC,Oversampling/DC,Oversampling/DC,Oversampling/DC
      mask Display:
      | port_label('output', 1, 'Ch.1')
      | port_label('output', 2, 'Ch.2')
  EL4xxx_0 : S-Function  FunctionName=ec_slave3  Parameters=Address,rv.SlaveConfig,rv.PortConfig,debug,tsample  SFunctionModules='ecrt_support'  EnableBusSupport=off  mask(EL4xxx){master=0, index=1, model=EL4002, vector=on, scale=, tsample=-1, debug=0, dc_mode=Free Run, dc_assign_activate=hex2dec('700'), dc_cycle0=0, dc_cycle0_factor=1, dc_shift0=0, dc_shift0_factor=0, dc_shift0_input=off, dc_cycle1=0, dc_cycle1_factor=1, dc_shift1=10000, dc_shift1_factor=0}
      mask prompts: index "Slave Index"; model "Device Model"; vector "Vector Input"; scale "Input Scale (empty for none)"; tsample "Sample Time (-1 for inherited)"; dc_mode "Distributed Clocks"; dc_assign_activate "Assign Activate"; dc_cycle0 "Cycle Time Sync 0"; dc_cycle0_factor "Factor"; dc_shift0 "Shift Time Sync0"; dc_shift0_factor "Factor"; dc_shift0_input "Shift Time0 Input"; dc_cycle1 "Cycle Time Sync1"; dc_cycle1_factor "Factor"; dc_shift1 "Shift Time Sync1"; dc_shift1_factor "Factor"
      mask help: Beckhoff Analog Output
      mask init:
      | Address = getEtherCATAddress(gcb, master, index, tsample);
      | 
      | rv = el4xxx.configure(model,vector,...
      |     EtherCATSlave.configureScale(2^15,scale),...
      |     [dc_mode, dc_assign_activate,...
      |      dc_cycle0, dc_cycle0_factor,...
      |      dc_shift0, dc_shift0_factor, dc_shift0_input,...
      |      dc_cycle1, dc_cycle1_factor,...
      |      dc_shift1, dc_shift1_factor]);
      mask Help:
      | This block generically implements the EtherCAT 16-Bit Analog Input Terminal for various models.
      | <p/>
      | The block input is generally a <tt>double</tt> from the range 0..1 for unipolar terminals and -1..1 for bipolar terminals, where 1 is the highest possible output of the terminal.
      | <p/>
      | Exceeding the input range simply saturates the terminal's output.
      | <p/>
      | The following Terminals are supported:
      | <center>
      | <table width="80%">
      | <tr><td>EL4008</td><td>0..10V Voltage Output</td></tr>
      | <tr><td>EL4028</td><td>4..20 mA Current Output</td></tr>
      | <tr><td>EL4034</td><td>-10..10V Voltage Output</td></tr>
      | <tr><td>EL4102</td><td>0..10V Voltage Output</td></tr>
      | <tr><td>EL4112</td><td>0..20mA Current Output</td></tr>
      | <tr><td>EL4122</td><td>4..20mA Current Output</td></tr>
      | <tr><td>EL4132</td><td>-10..10V Voltage Output</td></tr>
      | </table>
      | </center>
      | <p/>
      | Choose and set the following options:
      | <h4>Master:</h4>
      | Set the EtherCAT Master of this terminal.
      | 
      | <h4>Slave Index:</h4>
      | Set the EtherCAT slave index. Following address formats are allowed:
      | <ol>
      | <li> Absolute addressing: a scalar number <<b><tt>n</tt></b>> representing the (zero based) absolute position in the bus.
      | <li> SSId addressing: the Secondary Slave (or 'Alias') Addressing has the form <<b><tt>[alias position]</tt></b>> where <b><tt>alias</tt></b> is the Secondary Slave Id of the EtherCAT slave and <b><tt>position</tt></b> is the offset after the slave with the given <b><tt>alias</tt></b>. The SSId has to be preprogrammed into the slave with other service tools (see 'ethercat alias --help').
      | </ol>
      | 
      | <h4>Device Model:</h4>
      | Choose the device at the Indexed position of the master.
      | 
      | <h4>Input Type:</h4>
      | <ul>
      | <li>Choose <b>Vector Input</b> to have a single input as a vector
      | with a size corresponding to the channel count of the terminal. This mode also allows a control input and a status output port to be displayed.
      | <li>Choose <b>Separate Inputs</b> to have one input for every channel.
      | </ul>
      | 
      | <p>
      | Choosing <b>Status Output</b> provides a port of type <tt>uint8_T</tt> where the status is presented. This is only enabled when <b>Vector Output</b> is selected. Note: at the time of writing (1.2.2006) the terminals do not have a status output, and hence this option is disabled!
      | 
      | <p>
      | All input signals are multiplied with the factor <b>Input Scale</b>.
      | 
      | <p>
      | Set the <b>Sample Time</b> for the block. <tt>0</tt> is continuous sample time (runs at the model's base rate). Setting <tt>-1</tt> will try to set the time using back propagation.
      mask StyleString: edit,edit,popup(EL4001|EL4002|EL4004|EL4008|EL4011|EL4012|EL4014|EL4018|EL4021|EL4022|EL4024|EL4028|EL4031|EL4032|EL4034|EL4038|EL4102|EL4104|EL4112|EL4112-0010|EL4114|EL4122|EL4124|EL4132|EL4134),checkbox,edit,edit,edit,popup(Free Run|DC-Synchron|Custom),edit,min,max,min,max,checkbox,min,max,min,max
      mask CallbackString: |||||||EtherCATSlaveBlock().updateCustomDCEnable()||||||||||
      mask TabNameString: Main,Main,Main,Main,Main,Main,Main,Distributed Clocks,Distributed Clocks,Distributed Clocks,Distributed Clocks,Distributed Clocks,Distributed Clocks,Distributed Clocks,Distributed Clocks,Distributed Clocks,Distributed Clocks,Distributed Clocks
      mask Display:
      | fprintf('%s\n%s AIn\nM:%i Idx:%s', ...
      |     model, rv.function, master, mat2str(index))
  EL500x_0 : S-Function  LoadFcn=el500x('check')  FunctionName=ec_slave3  Parameters=Address,rv.SlaveConfig,rv.PortConfig,debug,tsample  SFunctionModules='ecrt_support'  EnableBusSupport=off  mask(EL500x){master=0, index=1, model=EL5001, code1=Binary, baud1=1250k, frame1=Multiturn (25 bits), fsize1=25, length1=24, frame_error1=off, power_fail1=off, inh_time1=0, code2=Binary, baud2=1250k, frame2=Multiturn (25 bits), fsize2=25, length2=24, frame_error2=off, power_fail2=off, inh_time2=0, frame_size=off, timestamp=off, dcmode=FreeRun/SM-Synchron, dccustom=[hex2dec('700'),0,1,0,0,0,0,1,15000,0], tsample=0, debug=0}
      mask prompts: index "Slave Index"; model "Device Model"; code1 "SSI Code (CoE #x80n0:6)"; baud1 "Baudrate (CoE #x80n0:9)"; frame1 "Frame Type (CoE #x80n0:f)"; fsize1 "SSI Frame Size (CoE #x80n0:11)"; length1 "Data Length (CoE #x80n0:12)"; frame_error1 "Disable Frame Error (CoE #x80n0:1)"; power_fail1 "Enable Power Failure bit (CoE #x80n0:2)"; inh_time1 "Min Inhibit Time [us] (0 = disabled) (CoE #x80n0:13)"; code2 "SSI Code (CoE #x80n0:6)"; baud2 "Baudrate (CoE #x80n0:9)"; frame2 "Frame Type (CoE #x80n0:f)"; fsize2 "SSI Frame Size (CoE #x80n0:11)"; length2 "Data Length (CoE #x80n0:12)"; frame_error2 "Disable Frame Error (CoE #x80n0:1)"; power_fail2 "Enable Power Failure bit (CoE #x80n0:2)"; inh_time2 "Min Inhibit Time [us] (0 = disabled) (CoE #x80n0:13)"; frame_size "Check SSI frame size (CoE #x8000:5)"; timestamp "Timestamp (PDO #x1a02)"; dcmode "DC Mode"; dccustom "DC Customer"; tsample "Sample Time"
      mask help: Beckhoff EtherCAT SSI Input
      mask init:
      | masterStr = '';        
      | positionStr = '';      
      | [Address masterStr positionStr] = ...
      |     getEtherCATAddress(gcb, master, index, tsample);
      | 
      | rv = get_param(gcbh,'UserData');
      | count = numel(rv.SlaveConfig.sm{1}{3});
      | if rv.SlaveConfig.ssi_monitor
      |     rv.dc = {...
      |         hex2dec('8000'), 1, 8,frame_error1;...
      |         hex2dec('8000'), 2, 8,power_fail1;...
      |         hex2dec('8000'), 5, 8,frame_size;...
      |         hex2dec('8000'), 6, 8,code1;...
      |         hex2dec('8000'),15, 8,frame1-1;...
      |         hex2dec('8000'),17,16,fsize1;...
      |         hex2dec('8000'),18,16,length1;...
      |     };
      | elseif count == 1
      |     rv.dc = {...
      |         hex2dec('8010'), 1, 8,frame_error1;...
      |         hex2dec('8010'), 2, 8,power_fail1;...
      |         hex2dec('8010'), 3, 8,double(inh_time1 > 0);...
      |         hex2dec('8010'), 6, 8,code1;...
      |         hex2dec('8010'), 9, 8,baud1-1;...
      |         hex2dec('8010'),15, 8,frame1-1;...
      |         hex2dec('8010'),17,16,fsize1;...
      |         hex2dec('8010'),18,16,length1;...
      |         hex2dec('8010'),19,16,inh_time1;...
      |     };
      | else
      |     rv.dc = {...
      |         hex2dec('8000'), 1, 8,frame_error1;...
      |         hex2dec('8000'), 2, 8,power_fail1;...
      |         hex2dec('8000'), 3, 8,double(inh_time1 > 0);...
      |         hex2dec('8000'), 6, 8,code1;...
      |         hex2dec('8000'), 9, 8,baud1-1;...
      |         hex2dec('8000'),15, 8,frame1-1;...
      |         hex2dec('8000'),17,16,fsize1;...
      |         hex2dec('8000'),18,16,length1;...
      |         hex2dec('8000'),19,16,inh_time1;...
      |         hex2dec('8010'), 1, 8,frame_error2;...
      |         hex2dec('8010'), 2, 8,power_fail2;...
      |         hex2dec('8010'), 3, 8,double(inh_time2 > 0);...
      |         hex2dec('8010'), 6, 8,code2;...
      |         hex2dec('8010'), 9, 8,baud2-1;...
      |         hex2dec('8010'),15, 8,frame2-1;...
      |         hex2dec('8010'),17,16,fsize2;...
      |         hex2dec('8010'),18,16,length2;...
      |         hex2dec('8010'),19,16,inh_time2;...
      |     };
      | end
      mask Help: web(etherlab_help_path('el500x.html'), '-helpbrowser');
      mask StyleString: edit,edit,popup(EL5001|EL5001-0011|EL5002),popup(Binary|Gray),popup(1250k|1000k|500k|250k|125k),popup(Multiturn (25 bits)|Singleturn (13 bits)|Variable (set size in Frame Size)),edit,edit,checkbox,checkbox,edit,popup(Binary|Gray),popup(1250k|1000k|500k|250k|125k),popup(Multiturn (25 bits)|Singleturn (13 bits)|Variable (set size in Frame Size)),edit,edit,checkbox,checkbox,edit,checkbox,checkbox,popup(FreeRun/SM-Synchron|DC-Synchron|DC-Synchron (input based)|DC-Latch active (only for EL5001-001x)|DC-Customized),edit,edit,edit
      mask CallbackString: ||el500x('set')|||el500x('ui')||||el500x('set')||||el500x('ui')||||el500x('set')|||el500x('set')|el500x('ui')|||
      mask TabNameString: Main,Main,Main,Chan1,Chan1,Chan1,Chan1,Chan1,Chan1,Chan1,Chan1,Chan2,Chan2,Chan2,Chan2,Chan2,Chan2,Chan2,Chan2,EL5001-001x,EL5001-001x,Main,Main,Main,Main
      mask Display:
      | fprintf('%s\nSSI Input\nM:%s Idx:%s', ...
      |     model, masterStr, positionStr)
  EL5021_0 : S-Function  FunctionName=ec_slave3  Parameters=Address,rv.SlaveConfig,rv.PortConfig,debug,tsample  SFunctionModules='ecrt_support'  EnableBusSupport=off  mask(EL5021){master=0, index=1, model=EL5021, tsample=-1, debug=0, dc_mode=FreeRun/SM-Synchron, dc_assign_activate=hex2dec('700'), dc_cycle0=[], dc_cycle0_factor=1, dc_shift0=-30600, dc_shift0_factor=[], dc_shift0_input=on, dc_cycle1=[], dc_cycle1_factor=1, dc_shift1=25000, dc_shift1_factor=[], x8000_01=off, x8000_0E=off, x8001_01=on, x8001_02=on, x8001_11=10}
      mask prompts: index "Slave Index"; model "Device Model"; tsample "Sample Time (-1 inherited)"; dc_mode "Mode"; dc_assign_activate "Assign Activate"; dc_cycle0 "Cycle Time Sync 0"; dc_cycle0_factor "Factor"; dc_shift0 "Shift Time Sync0"; dc_shift0_factor "Factor"; dc_shift0_input "Shift Time0 Input"; dc_cycle1 "Cycle Time Sync1"; dc_cycle1_factor "Factor"; dc_shift1 "Shift Time Sync1"; dc_shift1_factor "Factor"; x8000_01 "8000:01 - Enable C reset"; x8000_0E "8000:0E - Reversion of rotation"; x8001_01 "8001:01 - Frequency error counter"; x8001_02 "8001:02 - Amplitude error counter"; x8001_11 "8001:11 - Analog resolution"
      mask help: Beckhoff EtherCAT 1Ch. Sin/Cos Encoder
      mask init:
      | Address = getEtherCATAddress(gcb,master,index,tsample);
      | 
      | rv = el5021().configure(model,...
      |     [dc_mode, dc_assign_activate, ...
      |     dc_cycle0, dc_cycle0_factor,...
      |     dc_shift0, dc_shift0_factor, dc_shift0_input,...
      |     dc_cycle1, dc_cycle1_factor,...
      |     dc_shift1, dc_shift1_factor], ...
      |     [x8000_01, x8000_0E, x8001_01, x8001_02, x8001_11]);
      settings: AttributesFormatString=%<model>\nM:%<master> Idx:%<index>
      mask Help: web(etherlab_help_path('el5021.html'), '-helpbrowser');
      mask StyleString: edit,edit,popup(EL5021),edit,edit,popup(FreeRun/SM-Synchron|DC-Synchron|DC-Synchron (input based)|Custom),edit,min,max,min,max,checkbox,min,max,min,max,checkbox,checkbox,checkbox,checkbox,edit
      mask CallbackString: |||||EtherCATSlaveBlock(gcbh).updateCustomDCEnable();|||||||||||||||
      mask TabNameString: Main,Main,Main,Main,Main,Distributed Clocks,Distributed Clocks,Distributed Clocks,Distributed Clocks,Distributed Clocks,Distributed Clocks,Distributed Clocks,Distributed Clocks,Distributed Clocks,Distributed Clocks,Distributed Clocks,CoE #x800x,CoE #x800x,CoE #x800x,CoE #x800x,CoE #x800x
      mask Display:
      | port_label('input', 1, 'bool[2]')
      | port_label('input', 2, 'Ctr val')
      | port_label('output', 1, 'bool[5]')
      | port_label('output', 2, 'Ctr')
      | port_label('output', 3, 'Latch')
  EL5101_0 : S-Function  LoadFcn=el5101('check')  FunctionName=ec_slave3  Parameters=Address,rv.SlaveConfig,rv.PortConfig,debug,tsample  SFunctionModules='ecrt_support'  EnableBusSupport=off  mask(EL5101){master=0, index=1, model=EL5101, dcmode=FreeRun/SM-Synchron, x1601=off, x1602=off, x1603=on, x1A01=off, x1A02=off, x1A03=on, x1A04=off, x1A05=off, x1A06=off, x1A07=off, x1A08=off, tsample=0, debug=0, n8000_01=off, n8000_02=off, n8000_03=off, n8000_04=on, n8000_05=off, n8001_01=100, n8001_02=65535, x8010_01=off, x8010_02=off, x8010_03=off, x8010_04=Enable pos. gate, x8010_08=on, x8010_0A=off, x8010_0B=on, x8010_0C=on, x8010_0D=off, x8010_0E=off, x8010_10=on, x8010_11=10000, x8010_13=100, x8010_14=100, x8010_15=100, x8010_16=500, x8010_17=1600}
      mask prompts: index "Slave Index"; model "Device Model"; dcmode "DC Mode"; x1601 "RxPdo #x1601 (Excl 1602,1603)"; x1602 "RxPdo #x1602 (Excl 1601,1603)"; x1603 "RxPdo #x1603 (Excl 1601,1602)"; x1A01 "TxPdo #x1a01 (Excl 1a03,1a04,1a05,1a06,1a07,1a08)"; x1A02 "TxPdo #x1a02 (Excl 1a03,1a04,1a05,1a06,1a07,1a08)"; x1A03 "TxPdo #x1a03 (Excl 1a01,1a02,1a04)"; x1A04 "TxPdo #x1a04 (Excl 1a01,1a02,1a03)"; x1A05 "TxPdo #x1a05 (Excl 1a01,1a02,1a06)"; x1A06 "TxPdo #x1a06 (Excl 1a01,1a02,1a05)"; x1A07 "TxPdo #x1a07 (Excl 1a01,1a02,1a08)"; x1A08 "TxPdo #x1a08 (Excl 1a01,1a02,1a07)"; tsample "Sample Time (-1 inherited)"; n8000_01 "8000:01 - Enable Register Reload"; n8000_02 "8000:02 - Enable Index Reset"; n8000_03 "8000:03 - Enable FWD Count"; n8000_04 "8000:04 - Enable Positive Gate"; n8000_05 "8000:05 - Enable Negaitive Gate"; n8001_01 "8001:01 - Frequency Window"; n8001_02 "8001:02 - Counter Reload Value"; x8010_01 "8010:01 - Enable C reset"; x8010_02 "8010:02 - Enable extern reset"; x8010_03 "8010:03 - Enable up/down counter"; x8010_04 "8010:04 - Gate polarity"; x8010_08 "8010:08 - Disable filter"; x8010_0A "8010:0A - Enable micro increments"; x8010_0B "8010:0B - Open cct det A"; x8010_0C "8010:0C - Open cct det B"; x8010_0D "8010:0D - Open cct det C"; x8010_0E "8010:0E - Reversion of rotation"; x8010_10 "8010:10 - Extern Reset polarity"; x8010_11 "8010:11 - Frequency window"; x8010_13 "8010:13 - Frequency scaling"; x8010_14 "8010:14 - Period scaling"; x8010_15 "8010:15 - Frequency resolution"; x8010_16 "8010:16 - Period resolution"; x8010_17 "8010:17 - Frequency Wait Time"
      mask help: Beckhoff EtherCAT Incremental Encoder Input
      mask init:
      | masterStr = '';
      | positionStr = '';
      | [Address masterStr positionStr] = ...
      |     getEtherCATAddress(gcb,master,index,tsample);
      | 
      | el5101('set');
      | rv = get_param(gcbh,'UserData');
      | rv.SlaveConfig.sdo = {...
      |     hex2dec('1011'), 1,32,hex2dec('64616f6c');
      |     hex2dec('8000'), 1, 8,n8000_01;
      |     hex2dec('8000'), 2, 8,n8000_02;
      |     hex2dec('8000'), 3, 8,n8000_03;
      |     hex2dec('8000'), 4, 8,n8000_04;
      |     hex2dec('8000'), 5, 8,n8000_05;
      |     hex2dec('8001'), 1,16,n8001_01;
      |     hex2dec('8001'), 2,16,n8001_02;
      |     hex2dec('8010'), 1, 8,x8010_01;
      |     hex2dec('8010'), 2, 8,x8010_02;
      |     hex2dec('8010'), 3, 8,x8010_03;
      |     hex2dec('8010'), 4, 8,x8010_04-1;
      |     hex2dec('8010'), 8, 8,x8010_08;
      |     hex2dec('8010'),10, 8,x8010_0A;
      |     hex2dec('8010'),11, 8,x8010_0B;
      |     hex2dec('8010'),12, 8,x8010_0C;
      |     hex2dec('8010'),13, 8,x8010_0D;
      |     hex2dec('8010'),14, 8,x8010_0E;
      |     hex2dec('8010'),16, 8,x8010_10;
      |     hex2dec('8010'),17,16,x8010_11;
      |     hex2dec('8010'),19,16,x8010_13;
      |     hex2dec('8010'),20,16,x8010_14;
      |     hex2dec('8010'),21,16,x8010_15;
      |     hex2dec('8010'),22,16,x8010_16;
      |     hex2dec('8010'),23,16,x8010_17;
      | };
      mask Help: web(etherlab_help_path('el5101.html'), '-helpbrowser');
      mask StyleString: edit,edit,popup(EL5101|EL5101-1006),popup(FreeRun/SM-Synchron|DC-Synchron|DC-Synchron (input based)),checkbox,checkbox,checkbox,checkbox,checkbox,checkbox,checkbox,checkbox,checkbox,checkbox,checkbox,edit,edit,checkbox,checkbox,checkbox,checkbox,checkbox,edit,edit,checkbox,checkbox,checkbox,popup(Disable gate|Enable pos. gate|Enable neg. gate),checkbox,checkbox,checkbox,checkbox,checkbox,checkbox,checkbox,edit,edit,edit,edit,edit,edit
      mask CallbackString: ||||el5101('ui')|el5101('ui')|el5101('ui')|el5101('ui')|el5101('ui')|el5101('ui')|el5101('ui')|el5101('ui')|el5101('ui')|el5101('ui')|el5101('ui')||||||||||||||||||||||||||
      mask TabNameString: Main,Main,Main,Main,Main,Main,Main,Main,Main,Main,Main,Main,Main,Main,Main,Main,Main,CoE #x8000,CoE #x8000,CoE #x8000,CoE #x8000,CoE #x8000,CoE #x8001,CoE #x8001,CoE #x8010,CoE #x8010,CoE #x8010,CoE #x8010,CoE #x8010,CoE #x8010,CoE #x8010,CoE #x8010,CoE #x8010,CoE #x8010,CoE #x8010,CoE #x8010,CoE #x8010,CoE #x8010,CoE #x8010,CoE #x8010,CoE #x8010
      mask Display:
      | fprintf('%s\nIncr.-Enc\nM:%s Idx:%s',...
      |     model, masterStr, positionStr)
  EL5101_0010_0 : S-Function  LoadFcn=el5101_0010('check')  FunctionName=ec_slave3  Parameters=Address,rv.SlaveConfig,rv.PortConfig,debug,tsample  SFunctionModules='ecrt_support'  EnableBusSupport=off  mask(EL5101-0010){master=0, index=1, model=EL5101-0010, dcmode=FreeRun/SM-Synchron, x1600=on, x1601=off, x1A00=on, x1A01=off, x1A02=off, x1A03=off, x1A04=off, x1A05=off, tsample=0, debug=0, x8000_01=off, x8000_02=off, x8000_04=Enable pos. gate, x8000_0B=on, x8000_0C=on, x8000_0D=off, x8000_0E=off, x8000_10=on, x8000_11=10000, x8000_13=100, x8000_14=100, x8000_15=100, x8000_16=100, x8000_17=400}
      mask prompts: index "Slave Index"; model "Device Model"; dcmode "DC Mode"; x1600 "RxPdo #x1600 (Excl 1601)"; x1601 "RxPdo #x1601 (Excl 1600)"; x1A00 "TxPdo #x1a00 (Excl 1a01)"; x1A01 "TxPdo #x1a01 (Excl 1a00)"; x1A02 "TxPdo #x1a02 (Excl 1a03)"; x1A03 "TxPdo #x1a03 (Excl 1a02)"; x1A04 "TxPdo #x1a04 (Excl 1a05)"; x1A05 "TxPdo #x1a05 (Excl 1a04)"; tsample "Sample Time (-1 inherited)"; x8000_01 "8000:01 - Enable C reset"; x8000_02 "8000:02 - Enable extern reset"; x8000_04 "8000:04 - Gate polarity"; x8000_0B "8000:0B - Open cct det A"; x8000_0C "8000:0C - Open cct det B"; x8000_0D "8000:0D - Open cct det C"; x8000_0E "8000:0E - Reversion of rotation"; x8000_10 "8000:10 - Extern Reset polarity"; x8000_11 "8000:11 - Frequency window"; x8000_13 "8000:13 - Frequency scaling"; x8000_14 "8000:14 - Period scaling"; x8000_15 "8000:15 - Frequency resolution"; x8000_16 "8000:16 - Period resolution"; x8000_17 "8000:17 - Frequency Wait Time"
      mask help: Beckhoff EtherCAT Incremental Encoder Input
      mask init:
      | masterStr = '';
      | positionStr = '';
      | [Address masterStr positionStr] = ...
      |     getEtherCATAddress(gcb,master,index,tsample);
      | 
      | el5101_0010('set');
      | rv = get_param(gcbh,'UserData');
      | rv.SlaveConfig.sdo = {...
      |     hex2dec('1011'), 1,32,hex2dec('64616f6c');
      |     hex2dec('8000'), 1, 8,x8000_01;
      |     hex2dec('8000'), 2, 8,x8000_02;
      |     hex2dec('8000'), 4, 8,x8000_04-1;
      |     hex2dec('8000'),11, 8,x8000_0B;
      |     hex2dec('8000'),12, 8,x8000_0C;
      |     hex2dec('8000'),13, 8,x8000_0D;
      |     hex2dec('8000'),14, 8,x8000_0E;
      |     hex2dec('8000'),16, 8,x8000_10;
      |     hex2dec('8000'),17,16,x8000_11;
      |     hex2dec('8000'),19,16,x8000_13;
      |     hex2dec('8000'),20,16,x8000_14;
      |     hex2dec('8000'),21,16,x8000_15;
      |     hex2dec('8000'),22,16,x8000_16;
      |     hex2dec('8000'),23,16,x8000_17;
      | };
      mask Help: web(etherlab_help_path('el5101-0010.html'), '-helpbrowser');
      mask StyleString: edit,edit,popup(EL5101-0010),popup(FreeRun/SM-Synchron|DC-Synchron|DC-Synchron (input based)),checkbox,checkbox,checkbox,checkbox,checkbox,checkbox,checkbox,checkbox,edit,edit,checkbox,checkbox,popup(Disable gate|Enable pos. gate|Enable neg. gate),checkbox,checkbox,checkbox,checkbox,checkbox,edit,edit,edit,edit,edit,edit
      mask CallbackString: ||||el5101_0010('ui')|el5101_0010('ui')|el5101_0010('ui')|el5101_0010('ui')|el5101_0010('ui')|el5101_0010('ui')|el5101_0010('ui')|el5101_0010('ui')||||||||||||||||
      mask TabNameString: Main,Main,Main,Main,Main,Main,Main,Main,Main,Main,Main,Main,Main,Main,CoE #x8000,CoE #x8000,CoE #x8000,CoE #x8000,CoE #x8000,CoE #x8000,CoE #x8000,CoE #x8000,CoE #x8000,CoE #x8000,CoE #x8000,CoE #x8000,CoE #x8000,CoE #x8000
      mask Display:
      | fprintf('%s\nIncr.-Enc\nM:%s Idx:%s',...
      |     model, masterStr, positionStr)
  EL515x_1 : S-Function  LoadFcn=el515x('check')  FunctionName=ec_slave3  Parameters=Address,rv.SlaveConfig,rv.PortConfig,debug,tsample  SFunctionModules='ecrt_support'  EnableBusSupport=off  mask(EL515x){master=0, index=1, model=EL5152, dcmode=FreeRun/SM-Synchron, x1600=on, x1601=off, x1602=off, x1603=off, x1A00=on, x1A01=off, x1A02=off, x1A03=off, x1A04=off, x1A05=off, x1A06=off, x1A07=off, tsample=0, debug=0, x8000_01=off, x8000_02=off, x8000_03=off, x8000_04=Enable pos. gate, x8000_08=off, x8000_0A=off, x8000_0E=off, x8000_0F=off, x8000_10=on, x8000_11=10000, x8000_13=100, x8000_14=100, x8000_15=100, x8000_16=100, x8000_17=1600, x8010_03=off, x8010_08=off, x8010_0A=off, x8010_0E=off, x8010_0F=off, x8010_11=10000, x8010_13=100, x8010_14=100, x8010_15=100, x8010_16=100, x8010_17=1600}
      mask prompts: index "Slave Index"; model "Device Model"; dcmode "DC Mode"; x1600 "RxPdo #x1600 (Excl 1601)"; x1601 "RxPdo #x1601 (Excl 1600)"; x1602 "RxPdo #x1602 (Excl 1603)"; x1603 "RxPdo #x1603 (Excl 1602)"; x1A00 "TxPdo #x1a00 (Excl 1a01)"; x1A01 "TxPdo #x1a01 (Excl 1a00)"; x1A02 "TxPdo #x1a02 (Excl 1a03)"; x1A03 "TxPdo #x1a03 (Excl 1a02)"; x1A04 "TxPdo #x1a04 (Excl 1a05)"; x1A05 "TxPdo #x1a05 (Excl 1a04)"; x1A06 "TxPdo #x1a06 (Excl 1a07)"; x1A07 "TxPdo #x1a07 (Excl 1a06)"; tsample "Sample Time (-1 inherited)"; x8000_01 "8000:01 - Enable C reset"; x8000_02 "8000:02 - Enable extern reset"; x8000_03 "8000:03 - Enable up/down counter"; x8000_04 "8000:04 - Gate polarity"; x8000_08 "8000:08 - Disable filter"; x8000_0A "8000:0A - Enable micro increments"; x8000_0E "8000:0E - Reversion of rotation"; x8000_0F "8000:0F - Freqency window in ms"; x8000_10 "8000:10 - Extern Reset polarity"; x8000_11 "8000:11 - Frequency window"; x8000_13 "8000:13 - Frequency scaling"; x8000_14 "8000:14 - Period scaling"; x8000_15 "8000:15 - Frequency resolution"; x8000_16 "8000:16 - Period resolution"; x8000_17 "8000:17 - Frequency Wait Time"; x8010_03 "8010:03 - Enable up/down counter"; x8010_08 "8010:08 - Disable filter"; x8010_0A "8010:0A - Enable micro increments"; x8010_0E "8010:0E - Reversion of rotation"; x8010_0F "8010:0F - Freqency window in ms"; x8010_11 "8010:11 - Frequency window"; x8010_13 "8010:13 - Frequency scaling"; x8010_14 "8010:14 - Period scaling"; x8010_15 "8010:15 - Frequency resolution"; x8010_16 "8010:16 - Period resolution"; x8010_17 "8010:17 - Frequency Wait Time"
      mask help: Beckhoff EtherCAT Incremental Encoder Input
      mask init:
      | masterStr = '';
      | positionStr = '';
      | [Address masterStr positionStr] = ...
      |     getEtherCATAddress(gcb,master,index,tsample);
      | 
      | el515x('set');
      | rv = get_param(gcbh,'UserData');
      | rv.SlaveConfig.sdo = {...
      |     hex2dec('8000'), 3, 8,x8000_03;
      |     hex2dec('8000'), 8, 8,x8000_08;
      |     hex2dec('8000'),10, 8,x8000_0A;
      |     hex2dec('8000'),14, 8,x8000_0E;
      |     hex2dec('8000'),15, 8,x8000_0F;
      |     hex2dec('8000'),17,16,x8000_11;
      |     hex2dec('8000'),19,16,x8000_13;
      |     hex2dec('8000'),20,16,x8000_14;
      |     hex2dec('8000'),21,16,x8000_15;
      |     hex2dec('8000'),22,16,x8000_16;
      |     hex2dec('8000'),23,16,x8000_17;
      | };
      | 
      | if strncmp(model,'EL5151',6)
      |     rv.SlaveConfig.sdo = vertcat(rv.SlaveConfig.sdo,...
      |         { hex2dec('8000'), 1, 8,x8000_01;
      |           hex2dec('8000'), 2, 8,x8000_02;
      |           hex2dec('8000'), 4, 8,x8000_04;
      |           hex2dec('8000'),16, 8,x8000_10});
      | else
      |     rv.SlaveConfig.sdo = vertcat(rv.SlaveConfig.sdo,...
      |         { hex2dec('8010'), 3, 8,x8010_03;
      |           hex2dec('8010'), 8, 8,x8010_08;
      |           hex2dec('8010'),10, 8,x8010_0A;
      |           hex2dec('8010'),14, 8,x8010_0E;
      |           hex2dec('8010'),15, 8,x8010_0F;
      |           hex2dec('8010'),17,16,x8010_11;
      |           hex2dec('8010'),19,16,x8010_13;
      |           hex2dec('8010'),20,16,x8010_14;
      |           hex2dec('8010'),21,16,x8010_15;
      |           hex2dec('8010'),22,16,x8010_16;
      |           hex2dec('8010'),23,16,x8010_17});
      | end
      mask Help: web(etherlab_help_path('el515x.html'), '-helpbrowser');
      mask StyleString: edit,edit,popup(EL5151|EL5151-0080|EL5152),popup(FreeRun/SM-Synchron|DC-Synchron|DC-Synchron (input based)),checkbox,checkbox,checkbox,checkbox,checkbox,checkbox,checkbox,checkbox,checkbox,checkbox,checkbox,checkbox,edit,edit,checkbox,checkbox,checkbox,popup(Disable gate|Enable pos. gate|Enable neg. gate),checkbox,checkbox,checkbox,checkbox,checkbox,edit,edit,edit,edit,edit,edit,checkbox,checkbox,checkbox,checkbox,checkbox,edit,edit,edit,edit,edit,edit
      mask CallbackString: ||el515x('ui')||el515x('ui')|el515x('ui')|el515x('ui')|el515x('ui')|el515x('ui')|el515x('ui')|el515x('ui')|el515x('ui')|el515x('ui')|el515x('ui')|el515x('ui')|el515x('ui')||||||||||||||||||||||||||||
      mask TabNameString: Main,Main,Main,Main,Main,Main,Main,Main,Main,Main,Main,Main,Main,Main,Main,Main,Main,Main,CoE #x8000,CoE #x8000,CoE #x8000,CoE #x8000,CoE #x8000,CoE #x8000,CoE #x8000,CoE #x8000,CoE #x8000,CoE #x8000,CoE #x8000,CoE #x8000,CoE #x8000,CoE #x8000,CoE #x8000,CoE #x8010,CoE #x8010,CoE #x8010,CoE #x8010,CoE #x8010,CoE #x8010,CoE #x8010,CoE #x8010,CoE #x8010,CoE #x8010,CoE #x8010
      mask Display:
      | fprintf('%s\nIncr.-Enc\nM:%s Idx:%s',...
      |     model, masterStr, positionStr)
  EL515x_2 : S-Function  FunctionName=ec_slave3  Parameters=Address,rv.SlaveConfig,rv.PortConfig,debug,tsample  SFunctionModules='ecrt_support'  EnableBusSupport=off  mask(EL515x){master=0, index=1, model=EL5152, x1600=off, x1601=off, x1602=off, x1603=off, x1A00=on, x1A01=off, x1A02=off, x1A03=off, x1A04=off, x1A05=off, x1A06=off, x1A07=off, tsample=0, debug=0, dc_mode=FreeRun/SM-Synchron, dc_assign_activate=hex2dec('320')    % EL5151-x: '320'; El5152: '720', dc_cycle0=0, dc_cycle0_factor=1, dc_shift0=0, dc_shift0_factor=0, dc_shift0_input=off, dc_cycle1=0, dc_cycle1_factor=1, dc_shift1=0, dc_shift1_factor=0, x8000_01=off, x8000_02=off, x8000_03=off, x8000_04=Disable gate, x8000_08=off, x8000_0A=off, x8000_0E=off, x8000_0F=off, x8000_10=on, x8000_11=10000, x8000_13=100, x8000_14=100, x8000_15=100, x8000_16=100, x8000_17=1600, x8010_03=off, x8010_08=off, x8010_0A=off, x8010_0E=off, x8010_0F=off, x8010_11=10000, x8010_13=100, x8010_14=100, x8010_15=100, x8010_16=100, x8010_17=1600}
      mask prompts: index "Slave Index"; model "Device Model"; x1600 "RxPdo #x1600 (Excl 1601)"; x1601 "RxPdo #x1601 (Excl 1600)"; x1602 "RxPdo #x1602 (Excl 1603)"; x1603 "RxPdo #x1603 (Excl 1602)"; x1A00 "TxPdo #x1a00 (Excl 1a01)"; x1A01 "TxPdo #x1a01 (Excl 1a00)"; x1A02 "TxPdo #x1a02 (Excl 1a03)"; x1A03 "TxPdo #x1a03 (Excl 1a02)"; x1A04 "TxPdo #x1a04 (Excl 1a05)"; x1A05 "TxPdo #x1a05 (Excl 1a04)"; x1A06 "TxPdo #x1a06 (Excl 1a07)"; x1A07 "TxPdo #x1a07 (Excl 1a06)"; tsample "Sample Time (-1 inherited)"; dc_mode "DC Mode"; dc_assign_activate "Assign Activate"; dc_cycle0 "Cycle Time Sync 0 [ns]"; dc_cycle0_factor "Factor"; dc_shift0 "Shift Time Sync0 [ns]"; dc_shift0_factor "Factor"; dc_shift0_input "Shift Time0 Input"; dc_cycle1 "Cycle Time Sync1 [ns]"; dc_cycle1_factor "Factor"; dc_shift1 "Shift Time Sync1 [ns]"; dc_shift1_factor "Factor"; x8000_01 "8000:01 - Enable C reset"; x8000_02 "8000:02 - Enable extern reset"; x8000_03 "8000:03 - Enable up/down counter"; x8000_04 "8000:04 - Gate polarity"; x8000_08 "8000:08 - Disable filter"; x8000_0A "8000:0A - Enable micro increments"; x8000_0E "8000:0E - Reversion of rotation"; x8000_0F "8000:0F - Freqency window in ms"; x8000_10 "8000:10 - Extern Reset polarity"; x8000_11 "8000:11 - Frequency window"; x8000_13 "8000:13 - Frequency scaling"; x8000_14 "8000:14 - Period scaling"; x8000_15 "8000:15 - Frequency resolution"; x8000_16 "8000:16 - Period resolution"; x8000_17 "8000:17 - Frequency Wait Time"; x8010_03 "8010:03 - Enable up/down counter"; x8010_08 "8010:08 - Disable filter"; x8010_0A "8010:0A - Enable micro increments"; x8010_0E "8010:0E - Reversion of rotation"; x8010_0F "8010:0F - Freqency window in ms"; x8010_11 "8010:11 - Frequency window"; x8010_13 "8010:13 - Frequency scaling"; x8010_14 "8010:14 - Period scaling"; x8010_15 "8010:15 - Frequency resolution"; x8010_16 "8010:16 - Period resolution"; x8010_17 "8010:17 - Frequency Wait Time"
      mask help: Beckhoff EtherCAT Incremental Encoder Input
      mask init:
      | Address = getEtherCATAddress(gcb,master,index,tsample);
      | % 
      | % el515x('set');
      | % rv = get_param(gcbh,'UserData');
      | % rv.SlaveConfig.sdo = {...
      | %     hex2dec('8000'), 3, 8,x8000_03;
      | %     hex2dec('8000'), 8, 8,x8000_08;
      | %     hex2dec('8000'),10, 8,x8000_0A;
      | %     hex2dec('8000'),14, 8,x8000_0E;
      | %     hex2dec('8000'),15, 8,x8000_0F;
      | %     hex2dec('8000'),17,16,x8000_11;
      | %     hex2dec('8000'),19,16,x8000_13;
      | %     hex2dec('8000'),20,16,x8000_14;
      | %     hex2dec('8000'),21,16,x8000_15;
      | %     hex2dec('8000'),22,16,x8000_16;
      | %     hex2dec('8000'),23,16,x8000_17;
      | % };
      | % 
      | % if strncmp(model,'EL5151',6)
      | %     rv.SlaveConfig.sdo = vertcat(rv.SlaveConfig.sdo,...
      | %         { hex2dec('8000'), 1, 8,x8000_01;
      | %           hex2dec('8000'), 2, 8,x8000_02;
      | %           hex2dec('8000'), 4, 8,x8000_04;
      | %           hex2dec('8000'),16, 8,x8000_10});
      | % else
      | %     rv.SlaveConfig.sdo = vertcat(rv.SlaveConfig.sdo,...
      | %         { hex2dec('8010'), 3, 8,x8010_03;
      | %           hex2dec('8010'), 8, 8,x8010_08;
      | %           hex2dec('8010'),10, 8,x8010_0A;
      | %           hex2dec('8010'),14, 8,x8010_0E;
      | %           hex2dec('8010'),15, 8,x8010_0F;
      | %           hex2dec('8010'),17,16,x8010_11;
      | %           hex2dec('8010'),19,16,x8010_13;
      | %           hex2dec('8010'),20,16,x8010_14;
      | %           hex2dec('8010'),21,16,x8010_15;
      | %           hex2dec('8010'),22,16,x8010_16;
      | %           hex2dec('8010'),23,16,x8010_17});
      | % end
      mask Help: web(etherlab_help_path('el515x.html'), '-helpbrowser');
      mask StyleString: edit,edit,popup(EL5151|EL5151-0080|EL5152),checkbox,checkbox,checkbox,checkbox,checkbox,checkbox,checkbox,checkbox,checkbox,checkbox,checkbox,checkbox,edit,edit,popup(FreeRun/SM-Synchron|DC-Synchron|DC-Synchron (input based)|Custom),edit,min,max,min,max,checkbox,min,max,min,max,checkbox,checkbox,checkbox,popup(Disable gate|Enable pos. gate|Enable neg. gate),checkbox,checkbox,checkbox,checkbox,checkbox,edit,edit,edit,edit,edit,edit,checkbox,checkbox,checkbox,checkbox,checkbox,edit,edit,edit,edit,edit,edit
      mask CallbackString: |||||||||||||||||EtherCATSlaveBlock(gcbh).updateCustomDCEnable();||||||||||||||||||||||||||||||||||||
      mask TabNameString: Main,Main,Main,Main,Main,Main,Main,Main,Main,Main,Main,Main,Main,Main,Main,Main,Main,Distributed Clocks,Distributed Clocks,Distributed Clocks,Distributed Clocks,Distributed Clocks,Distributed Clocks,Distributed Clocks,Distributed Clocks,Distributed Clocks,Distributed Clocks,Distributed Clocks,CoE #x8000,CoE #x8000,CoE #x8000,CoE #x8000,CoE #x8000,CoE #x8000,CoE #x8000,CoE #x8000,CoE #x8000,CoE #x8000,CoE #x8000,CoE #x8000,CoE #x8000,CoE #x8000,CoE #x8000,CoE #x8010,CoE #x8010,CoE #x8010,CoE #x8010,CoE #x8010,CoE #x8010,CoE #x8010,CoE #x8010,CoE #x8010,CoE #x8010,CoE #x8010
      mask Display: fprintf('%s\nIncr.-Enc\nM:%i Idx:%s', model, master, mat2str(index))
  EL9xxx_0 : S-Function  FunctionName=ec_slave3  Parameters=Address,rv.SlaveConfig,rv.PortConfig,debug,tsample  SFunctionModules='ecrt_support'  EnableBusSupport=off  mask(EL9xxx){master=0, index=1, model=EL9110, vector=off, tsample=0, debug=0}
      mask prompts: index "Slave Index"; model "Device Model"; vector "Vector Outputs"; tsample "Sample Time"; debug "Debug Level"
      mask help:
      | Beckhoff EtherCAT System Terminals
      | with diagnosis
      mask init:
      | Address = getEtherCATAddress(gcb, master, index, tsample);
      | 
      | rv = el9xxx().configure(model,vector);
      |  
      | EtherCATSlaveBlock().setPortNames(...
      |     {}, {rv.PortConfig.output.portname});
      settings: AttributesFormatString=%<model>\nM:%<master> Idx:%<index>
      mask Help: web(etherlab_help_path('el9xxx.html'), '-helpbrowser');
      mask StyleString: edit,edit,popup(EL9110|EL9160|EL9210|EL9210-0020|EL9260|EL9410|EL9505|EL9508|EL9510|EL9512|EL9515|EL9560),checkbox,edit,edit
      mask Display: port_label('output', 1, 'Pwr OK')
  EP1xxx_0 : S-Function  FunctionName=ec_slave3  Parameters=Address,rv.SlaveConfig,rv.PortConfig,debug,tsample  SFunctionModules='ecrt_support'  EnableBusSupport=off  mask(EP1xxx){master=0, index=1, model=EP1008-0002, vector=on, tsample=0, debug=0}
      mask prompts: index "Slave Index"; model "Device Model"; vector "Vector Output"; tsample "Sample Time"; debug "Deug Level"
      mask help: Beckhoff EtherCAT Digital Input Fieldbus Box
      mask init:
      | Address = getEtherCATAddress(gcb, master, index, tsample);
      | 
      | rv = ep1xxx.configure(model,vector);
      mask Help:
      | This block implements the Beckhoff's EtherCAT series of Digital Input Terminals.
      | <p/>
      | Choose or set the following options:
      | <h4>Master:</h4>
      | Set the EtherCAT Master number that this terminal is connected to.
      | 
      | <h4>Slave Index:</h4>
      | Set the EtherCAT slave index. Following address formats are allowed:
      | <ol>
      | <li> Absolute addressing: a scalar number <<b><tt>n</tt></b>> representing the (zero based) absolute position in the bus.
      | <li> SSId addressing: the Secondary Slave (or 'Alias') Addressing has the form <<b><tt>[alias position]</tt></b>> where <b><tt>alias</tt></b> is the Secondary Slave Id of the EtherCAT slave and <b><tt>position</tt></b> is the offset after the slave with the given <b><tt>alias</tt></b>. The SSId has to be preprogrammed into the slave with other service tools (see 'ethercat alias --help').
      | </ol>
      | 
      | <h4> Device Model</h4>
      | Select the model that is used. This sets the number of outputs of this block.
      | 
      | <h4>Output Type</h4>
      | The block output type corresponding to the terminal inputs can be one of the following:
      | <ul>
      | <li><b>Vector Output</b>: This sets one output vector with a width equal to the number of digital inputs to the terminal.
      | <li><b>Separate Outputs</b>: This sets the number of outputs corresponding to the digital inputs to the terminal.
      | </ul>
      | 
      | <h4>Sample Time</h4>
      | Select the correct sample time. Setting this to 0 makes for a sample time at the model's base rate. If another block can set the sample time, choose -1 for inherited sample time.
      mask StyleString: edit,edit,popup(EP1008-0001|EP1008-0002|EP1018-0001|EP1018-0002|EP1111|EP1122-0001|EP1809-0021|EP1809-0022|EP1819-0022),checkbox,edit,edit
      mask Display: fprintf('%s\nM:%i Idx:%s', model, master, mat2str(index))
  EP2xxx_0 : S-Function  FunctionName=ec_slave3  Parameters=Address,rv.SlaveConfig,rv.PortConfig,debug,tsample  SFunctionModules='ecrt_support'  EnableBusSupport=off  mask(EP2xxx){master=0, index=1, model=EP2001-1000, vector=on, tsample=0, debug=0}
      mask prompts: index "Slave Index"; model "Device Model"; vector "Vector Input"; tsample "Sample Time"; debug "Debug Level"
      mask help: Beckhoff EtherCAT Digital Output Fieldbus Box
      mask init:
      | Address = getEtherCATAddress(gcb, master, index, tsample);
      | 
      | rv = ep2xxx.configure(model,vector);
      mask Help:
      | This block implements the Beckhoff's EtherCAT series of Digital Input Terminals.
      | <p/>
      | Choose or set the following options:
      | <h4>Master:</h4>
      | Set the EtherCAT Master number that this terminal is connected to.
      | 
      | <h4>Slave Index:</h4>
      | Set the EtherCAT slave index. Following address formats are allowed:
      | <ol>
      | <li> Absolute addressing: a scalar number <<b><tt>n</tt></b>> representing the (zero based) absolute position in the bus.
      | <li> SSId addressing: the Secondary Slave (or 'Alias') Addressing has the form <<b><tt>[alias position]</tt></b>> where <b><tt>alias</tt></b> is the Secondary Slave Id of the EtherCAT slave and <b><tt>position</tt></b> is the offset after the slave with the given <b><tt>alias</tt></b>. The SSId has to be preprogrammed into the slave with other service tools (see 'ethercat alias --help').
      | </ol>
      | 
      | <h4> Device Model</h4>
      | Select the model that is used. This sets the number of outputs of this block.
      | 
      | <h4>Output Type</h4>
      | The block output type corresponding to the terminal inputs can be one of the following:
      | <ul>
      | <li><b>Vector Output</b>: This sets one output vector with a width equal to the number of digital inputs to the terminal.
      | <li><b>Separate Outputs</b>: This sets the number of outputs corresponding to the digital inputs to the terminal.
      | </ul>
      | 
      | <h4>Sample Time</h4>
      | Select the correct sample time. Setting this to 0 makes for a sample time at the model's base rate. If another block can set the sample time, choose -1 for inherited sample time.
      mask StyleString: edit,edit,popup(EP2001-1000|EP2008-0001|EP2008-0002|EP2028-0001|EP2028-0002|EP2308-0000|EP2308-0001|EP2308-0002|EP2318-0001|EP2318-0002|EP2328-0001|EP2328-0002|EP2338-0001|EP2338-0002|EP2339-0021|EP2339-0022|EP2624|EP2624-0002|EP2809-0021|EP2809-0022),checkbox,edit,edit
      mask Display: fprintf('%s\nM:%i Idx:%s', model, master, mat2str(index))
  EP31xx_0 : S-Function  LoadFcn=|  FunctionName=ec_slave3  Parameters=Address,rv.SlaveConfig,rv.PortConfig,debug,tsample  SFunctionModules='ecrt_support'  EnableBusSupport=off  mask(EP3xxx){master=0, index=1, model=EP3174-0002, type_1=-10...+10 V, type_2=-10...+10 V, type_3=-10...+10 V, type_4=-10...+10 V, dc=FreeRun/SM-Synchron, dccustomer=[1 hex2dec('700') 0 0 0 0 0 0 0], vector=on, raw=off, scale=1, offset=0, tau=1, status=off, tsample=0, debug=0}
      | ep31xx('check')                              
      | if ~strcmp(bdroot(gcb),'etherlab_lib')       
      |    disp([gcb ' is obsolete. Please replace'])
      | end
      mask prompts: index "Slave Index"; model "Device Model"; type_1 "Channel 1 Type"; type_2 "Channel 2 Type"; type_3 "Channel 3 Type"; type_4 "Channel 4 Type"; dc "DC Mode"; dccustomer "Dc Customer"; vector "Vector Ports"; raw "Raw Bits"; scale "Output Scale (empty for none)"; offset "Output Offset (empty for none)"; tau "LPF Time Constant (sec)"; status "Status Output"; tsample "Sample Time (-1 for inherited)"
      mask help: Beckhoff Analog Input 16-Bit Fieldbus Box
      mask init:
      | masterStr = '';
      | positionStr = '';
      | [Address masterStr positionStr] = ...
      |     getEtherCATAddress(gcb, master, index, tsample);
      | 
      | ep31xx('set');  % Report errors
      | 
      | rv = get_param(gcbh,'UserData');
      mask Help:
      | This block generically implements the EtherCAT 16-Bit Analog Input Fieldbus box Terminal for various models.
      | <p/>
      | The block input is generally a <tt>double</tt> from the range 0..1 for unipolar terminals and -1..1 for bipolar terminals, where 1 is the highest possible output of the terminal.
      | <p/>
      | Exceeding the input range simply saturates the terminal's output.
      | <p/>
      | The following Terminals are supported:
      | <center>
      | <table width="80%">
      | <tr><td>EP3174</td><td>4 port differential input</td></tr>
      | <tr><td>EP3182</td><td>2 port single ended input</td></tr>
      | <tr><td>EP3184</td><td>4 port single ended input</td></tr>
      | </table>
      | </center>
      | <p/>
      | Choose and set the following options:
      | <h4>Master:</h4>
      | Set the EtherCAT Master of this terminal.
      | 
      | <h4>Slave Index:</h4>
      | Set the EtherCAT slave index. Following address formats are allowed:
      | <ol>
      | <li> Absolute addressing: a scalar number <<b><tt>n</tt></b>> representing the (zero based) absolute position in the bus.
      | <li> SSId addressing: the Secondary Slave (or 'Alias') Addressing has the form <<b><tt>[alias position]</tt></b>> where <b><tt>alias</tt></b> is the Secondary Slave Id of the EtherCAT slave and <b><tt>position</tt></b> is the offset after the slave with the given <b><tt>alias</tt></b>. The SSId has to be preprogrammed into the slave with other service tools (see 'ethercat alias --help').
      | </ol>
      | 
      | <h4>Device Model:</h4>
      | Choose the device at the Indexed position of the master.
      | 
      | <h4>Channel 1-4 Type:</h4>
      | Choose the output type of the channel.
      | 
      | <h4>DC Mode:</h4>
      | Choose the DC Mode for the module.
      | 
      | <h4>DC Customer:</h4>
      | Do customized DC Settings in a vector
      | <<b><tt>[AssignActivate, CycleTimeSync0, CycleTimeSync0Factor, ShiftTimeSync0, ShiftTimeSync0Factor, ...
      | ShiftTimeSync0Input, CycleTimeSync1, CycleTimeSync1Factor, ShiftTimeSync1, ShiftTimeSync1Factor]</tt></b>>
      | 
      | <ul>
      | <li><<b><tt>AssignActivate:</tt></b>> Value for DC-mode setting
      | <li><<b><tt>CycleTimeSync0:</tt></b>> CycleTimeSync0 Value
      | <li><<b><tt>CycleTimeSync0Factor:</tt></b>> 1 or 0. If CycleTimeSync0Factor equals one the cycletimesync0 value is internally set to the process cycletime.
      | <li><<b><tt>ShiftTimeSync0:</tt></b>> ShiftTimeSync0 Value
      | <li><<b><tt>ShiftTimeSync0Factor:</tt></b>> 1 or 0. If ShiftTimeSync0Factor equals one the Slave is synced on the input event
      | <li><<b><tt>ShiftTimeSync0Input:</tt></b>> 1 or 0. If ShiftTimeSync0Input equals one the Slave is synced on the input event
      | <li><<b><tt>CycleTimeSync1:</tt></b>> CycleTimeSync1 Value
      | <li><<b><tt>CycleTimeSync1Factor:</tt></b>> 1 or 0. If CycleTimeSync1Factor equals one the CycletTimesSync1 value is internally set to the process cycletime.
      | <li><<b><tt>ShiftTimeSync1:</tt></b>>ShiftTimeSync1 Value
      | <li><<b><tt>ShiftTimeSync1Factor:</tt></b>> ShiftTimeSync1Factor Value
      | </ul>
      | 
      | <h4>Output Type:</h4>
      | <ul>
      | <li>Choose <b>Vector Output</b> to have a single output as a vector
      | with a size corresponding to the channel count of the terminal. This mode also allows a status output port to be displayed. <br/>
      | <li>Choose <b>Separate Outputs</b> to have one output for every channel.
      | </ul>
      | <h4>Output Full Scale</h4>
      | When <b>Output Data Type</b> is set to <b>Double with scale and offset</b>, the block's output value at full scale terminal input can be set here.
      | 
      | <h4>Output Offset</h4>
      | When <b>Output Data Type</b> is set to <b>Double with scale and offset</b>, the blocks output at zero terminal input can be set here. Note that the Full Scale above is also increased by this amount. Note furthermore that this corresponds to the minimum input for terminals such as 4..20mA.
      | 
      | <h4>Output Data Type</h4>
      | Choose the block's output data type for the output signal. Available are:
      | <ul>
      | <li><b><tt>Raw</tt></b> outputting the internal raw value as <tt>int16_T</tt> or <tt>uint16_T</tt> as appropriate
      | <li><b><tt>Double</tt></b> outputting 0..10, -10..10, 0..0.02 and 0.004..0.02 depending on the Model as appropriate
      | <li><b><tt>Double with scale and offset</tt></b>, allowing the output to be scaled with an offset.
      | </ul>
      | 
      | <p>
      | Choosing <b>Status Output</b> provides a port of type <tt>uint8_T</tt> where the status is presented. This is only enabled when <b>Vector Output</b> is selected. Terminal input over- and underrange can be detected using this output. See the terminal's documentation.
      | 
      | <h4>Output Filter</h4>
      | When not in <b>Raw</b> mode, the <b>Output Filter</b> checkbox becomes available, allowing the use of an internal low pass filter. Enter the <b>LPF Time Constant</b> for the filter in the field below.
      | <br>For continuous sample time systems (0 in Sample Time), the filter is also continuous. Discrete samples systems (Sample Time > 0) uses an equivalent discrete low pass filter with a similar time constant.
      | 
      | <p>
      | Set the <b>Sample Time</b> for the block. <tt>0</tt> is continuous sample time (runs at the model's base rate). Setting <tt>-1</tt> will try to set the time using back propagation.
      mask StyleString: edit,edit,popup(EP3174-0002|EP3182-1002|EP3184-0002|EP3184-1002),popup(-10...+10 V|0...20 mA|4...20 mA|0...10 V),popup(-10...+10 V|0...20 mA|4...20 mA|0...10 V),popup(-10...+10 V|0...20 mA|4...20 mA|0...10 V),popup(-10...+10 V|0...20 mA|4...20 mA|0...10 V),popup(FreeRun/SM-Synchron|DC-Synchron|DC-Synchron (input based)|DC-Customized),edit,checkbox,checkbox,edit,edit,edit,checkbox,edit,edit
      mask CallbackString: ||ep31xx('set');|||||ep31xx('set');||ep31xx('set');|||||||
      mask Display: fprintf('%s\nM:%i Idx:%s', model, master, mat2str(index));
  EP31xx_1 : S-Function  FunctionName=ec_slave3  Parameters=Address,rv.SlaveConfig,rv.PortConfig,debug,tsample  SFunctionModules='ecrt_support'  EnableBusSupport=off  mask(EP31xx){master=0, index=1, model=EP3182-1002, type_1=-10...+10 V, type_2=-10...+10 V, type_3=-10...+10 V, type_4=-10...+10 V, filter=Off, vector=on, status=on, gain=, offset=, tau=, tsample=0, debug=, dc_mode=FreeRun/SM-Synchron, dc_assign_activate=hex2dec('700'), dc_cycle0=0, dc_cycle0_factor=1, dc_shift0=0, dc_shift0_factor=0, dc_shift0_input=off, dc_cycle1=0, dc_cycle1_factor=1, dc_shift1=20000, dc_shift1_factor=0}
      mask prompts: index "Slave Index"; model "Device Model"; type_1 "Channel 1 Type"; type_2 "Channel 2 Type"; type_3 "Channel 3 Type"; type_4 "Channel 4 Type"; vector "Vector Ports"; status "Status Output"; gain "Output Scale (empty for none)"; offset "Output Offset (empty for none)"; tau "LPF Time Constant (sec)"; tsample "Sample Time (-1 for inherited)"; dc_mode "DC Mode"; dc_assign_activate "Assign Activate"; dc_cycle0 "Cycle Time Sync 0"; dc_cycle0_factor "Factor"; dc_shift0 "Shift Time Sync0"; dc_shift0_factor "Factor"; dc_shift0_input "Shift Time0 Input"; dc_cycle1 "Cycle Time Sync1"; dc_cycle1_factor "Factor"; dc_shift1 "Shift Time Sync1"; dc_shift1_factor "Factor"
      mask help: Beckhoff Analog Input 16-Bit Fieldbus Box
      mask init:
      | Address = getEtherCATAddress(gcb, master, index, tsample);
      | 
      | rv = ep31xx_1.configure(model,status,vector,...
      |     EtherCATSlave.configureScale(2^15,gain,offset,tau),...
      |     [dc_mode, dc_assign_activate, ...
      |      dc_cycle0, dc_cycle0_factor, ...
      |      dc_shift0, dc_shift0_factor, dc_shift0_input, ...
      |      dc_cycle1, dc_cycle1_factor, ...
      |      dc_shift1, dc_shift1_factor], ...
      |      filter, [type_1,type_2,type_3,type_4]);
      |  
      | if isfield(rv.PortConfig,'input')
      |     inputnames = {rv.PortConfig.input.portname};
      | else
      |     inputnames = {};
      | end
      | 
      | EtherCATSlaveBlock().setPortNames(inputnames,...
      |     {rv.PortConfig.output.portname})
      | 
      | set_param(gcb,'AttributesFormatString',...
      |     sprintf('%s\nM:%i Idx:%s',...
      |             model,master,mat2str(index)))
      settings: AttributesFormatString=|
      | EP3182-1002
      | M:0 Idx:1
      mask Help:
      | This block generically implements the EtherCAT 16-Bit Analog Input Fieldbus box Terminal for various models.
      | <p/>
      | The block input is generally a <tt>double</tt> from the range 0..1 for unipolar terminals and -1..1 for bipolar terminals, where 1 is the highest possible output of the terminal.
      | <p/>
      | Exceeding the input range simply saturates the terminal's output.
      | <p/>
      | The following Terminals are supported:
      | <center>
      | <table width="80%">
      | <tr><td>EP3174</td><td>4 port differential input</td></tr>
      | <tr><td>EP3182</td><td>2 port single ended input</td></tr>
      | <tr><td>EP3184</td><td>4 port single ended input</td></tr>
      | </table>
      | </center>
      | <p/>
      | Choose and set the following options:
      | <h4>Master:</h4>
      | Set the EtherCAT Master of this terminal.
      | 
      | <h4>Slave Index:</h4>
      | Set the EtherCAT slave index. Following address formats are allowed:
      | <ol>
      | <li> Absolute addressing: a scalar number <<b><tt>n</tt></b>> representing the (zero based) absolute position in the bus.
      | <li> SSId addressing: the Secondary Slave (or 'Alias') Addressing has the form <<b><tt>[alias position]</tt></b>> where <b><tt>alias</tt></b> is the Secondary Slave Id of the EtherCAT slave and <b><tt>position</tt></b> is the offset after the slave with the given <b><tt>alias</tt></b>. The SSId has to be preprogrammed into the slave with other service tools (see 'ethercat alias --help').
      | </ol>
      | 
      | <h4>Device Model:</h4>
      | Choose the device at the Indexed position of the master.
      | 
      | <h4>Channel 1-4 Type:</h4>
      | Choose the output type of the channel.
      | 
      | <h4>DC Mode:</h4>
      | Choose the DC Mode for the module.
      | 
      | <h4>DC Customer:</h4>
      | Do customized DC Settings in a vector
      | <<b><tt>[AssignActivate, CycleTimeSync0, CycleTimeSync0Factor, ShiftTimeSync0, ShiftTimeSync0Factor, ...
      | ShiftTimeSync0Input, CycleTimeSync1, CycleTimeSync1Factor, ShiftTimeSync1, ShiftTimeSync1Factor]</tt></b>>
      | 
      | <ul>
      | <li><<b><tt>AssignActivate:</tt></b>> Value for DC-mode setting
      | <li><<b><tt>CycleTimeSync0:</tt></b>> CycleTimeSync0 Value
      | <li><<b><tt>CycleTimeSync0Factor:</tt></b>> 1 or 0. If CycleTimeSync0Factor equals one the cycletimesync0 value is internally set to the process cycletime.
      | <li><<b><tt>ShiftTimeSync0:</tt></b>> ShiftTimeSync0 Value
      | <li><<b><tt>ShiftTimeSync0Factor:</tt></b>> 1 or 0. If ShiftTimeSync0Factor equals one the Slave is synced on the input event
      | <li><<b><tt>ShiftTimeSync0Input:</tt></b>> 1 or 0. If ShiftTimeSync0Input equals one the Slave is synced on the input event
      | <li><<b><tt>CycleTimeSync1:</tt></b>> CycleTimeSync1 Value
      | <li><<b><tt>CycleTimeSync1Factor:</tt></b>> 1 or 0. If CycleTimeSync1Factor equals one the CycletTimesSync1 value is internally set to the process cycletime.
      | <li><<b><tt>ShiftTimeSync1:</tt></b>>ShiftTimeSync1 Value
      | <li><<b><tt>ShiftTimeSync1Factor:</tt></b>> ShiftTimeSync1Factor Value
      | </ul>
      | 
      | <h4>Output Type:</h4>
      | <ul>
      | <li>Choose <b>Vector Output</b> to have a single output as a vector
      | with a size corresponding to the channel count of the terminal. This mode also allows a status output port to be displayed. <br/>
      | <li>Choose <b>Separate Outputs</b> to have one output for every channel.
      | </ul>
      | <h4>Output Full Scale</h4>
      | When <b>Output Data Type</b> is set to <b>Double with scale and offset</b>, the block's output value at full scale terminal input can be set here.
      | 
      | <h4>Output Offset</h4>
      | When <b>Output Data Type</b> is set to <b>Double with scale and offset</b>, the blocks output at zero terminal input can be set here. Note that the Full Scale above is also increased by this amount. Note furthermore that this corresponds to the minimum input for terminals such as 4..20mA.
      | 
      | <h4>Output Data Type</h4>
      | Choose the block's output data type for the output signal. Available are:
      | <ul>
      | <li><b><tt>Raw</tt></b> outputting the internal raw value as <tt>int16_T</tt> or <tt>uint16_T</tt> as appropriate
      | <li><b><tt>Double</tt></b> outputting 0..10, -10..10, 0..0.02 and 0.004..0.02 depending on the Model as appropriate
      | <li><b><tt>Double with scale and offset</tt></b>, allowing the output to be scaled with an offset.
      | </ul>
      | 
      | <p>
      | Choosing <b>Status Output</b> provides a port of type <tt>uint8_T</tt> where the status is presented. This is only enabled when <b>Vector Output</b> is selected. Terminal input over- and underrange can be detected using this output. See the terminal's documentation.
      | 
      | <h4>Output Filter</h4>
      | When not in <b>Raw</b> mode, the <b>Output Filter</b> checkbox becomes available, allowing the use of an internal low pass filter. Enter the <b>LPF Time Constant</b> for the filter in the field below.
      | <br>For continuous sample time systems (0 in Sample Time), the filter is also continuous. Discrete samples systems (Sample Time > 0) uses an equivalent discrete low pass filter with a similar time constant.
      | 
      | <p>
      | Set the <b>Sample Time</b> for the block. <tt>0</tt> is continuous sample time (runs at the model's base rate). Setting <tt>-1</tt> will try to set the time using back propagation.
      mask StyleString: edit,edit,popup(EP3174-0002|EP3182-1002|EP3184-0002|EP3184-1002),popup(-10...+10 V|0...20 mA|4...20 mA|0...10 V),popup(-10...+10 V|0...20 mA|4...20 mA|0...10 V),popup(-10...+10 V|0...20 mA|4...20 mA|0...10 V),popup(-10...+10 V|0...20 mA|4...20 mA|0...10 V),popup(Off|50Hz FIR|60Hz FIR|IIR 1|IIR 2|IIR 3|IIR 4|IIR 5|IIR 6|IIR 7|IIR 8),checkbox,checkbox,edit,edit,edit,edit,edit,popup(FreeRun/SM-Synchron|DC-Synchron|DC-Synchron (input based)|Custom),edit,min,max,min,max,checkbox,min,max,min,max
      mask CallbackString:
      | ||model = get_param(gcb,'model');
      | EtherCATSlaveBlock().setEnable({'type_3','type_4'},strcmp(model(6),'4'));|||||filter = ~strcmp(get_param(gcb,'filter'),'Off');
      | s = EtherCATSlaveBlock();
      | if filter
      |     set_param(gcb,'dc_mode','FreeRun/SM-Synchron');
      |     s.setEnable('dc_mode',false);
      | else
      |     s.setEnable('dc_mode',true);
      | end||||||||EtherCATSlaveBlock().updateCustomDCEnable()||||||||||
      mask TabNameString: Main,Main,Main,Main,Main,Main,Main,Main,Main,Main,Main,Main,Main,Main,Main,Distributed Clocks,Distributed Clocks,Distributed Clocks,Distributed Clocks,Distributed Clocks,Distributed Clocks,Distributed Clocks,Distributed Clocks,Distributed Clocks,Distributed Clocks,Distributed Clocks
      mask Display:
      | port_label('input', 1, 'DO')
      | port_label('output', 1, 'Value')
      | port_label('output', 2, 'Status')
  EP41xx_0 : S-Function  LoadFcn=ep41xx('check')  FunctionName=ec_slave3  Parameters=Address,rv.SlaveConfig,rv.PortConfig,debug,tsample  SFunctionModules='ecrt_support'  EnableBusSupport=off  mask(EP41xx){master=0, index=1, model=EP4174-0002, type_1=0...10 V, type_2=0...10 V, type_3=0...10 V, type_4=0...10 V, dcmode=FreeRun/SM-Synchron, dccustom=[hex2dec('730'),0,1,0,0,0,0,1,140000,0], vector=on, scale=, tsample=-1, debug=0}
      mask prompts: index "Slave Index"; model "Device Model"; type_1 "Channel 1 Type"; type_2 "Channel 2 Type"; type_3 "Channel 3 Type"; type_4 "Channel 4 Type"; dcmode "DC Mode"; dccustom "DC-Customized"; vector "Vector Input"; scale "Input Scale (empty for none)"; tsample "Sample Time (-1 for inherited)"
      mask help: Beckhoff Analog Output Fieldbus Box
      mask init:
      | masterStr = '';
      | positionStr = '';
      | [Address masterStr positionStr] = ...
      |     getEtherCATAddress(gcb, master, index, tsample);
      | 
      | ep41xx('set');  % Report errors
      | 
      | rv = get_param(gcbh,'UserData');
      | 
      | basetype = [type_1; type_2; type_3; type_4] - 1;
      | type_eq3 = basetype == 3;
      | basetype = basetype .* ~type_eq3 + type_eq3*6;
      | 
      | rowcount = numel(rv.SlaveConfig.sm{1}{3});
      | 
      | rv.SlaveConfig.sdo = num2cell(horzcat(...
      |     hex2dec('F800')*ones(rowcount,1),...
      |     (1:rowcount)',...
      |     16*ones(rowcount,1),...
      |     basetype));
      mask Help:
      | This block generically implements the EtherCAT 16-Bit Analog Input Terminal for various fieldbus boxes.
      | <p/>
      | The block input is generally a <tt>double</tt> from the range 0..1 for unipolar terminals and -1..1 for bipolar terminals, where 1 is the highest possible output of the terminal.
      | <p/>
      | Exceeding the input range simply saturates the terminal's output.
      | <p/>
      | The following Terminals are supported:
      | <center>
      | <table width="80%">
      | <tr><td>EP4174</td><td>+/-10V, 0..10V,  Voltage Output or 0..20mA, 4..20mA Current Output</td></tr>
      | </table>
      | </center>
      | <p/>
      | Choose and set the following options:
      | <h4>Master:</h4>
      | Set the EtherCAT Master of this terminal.
      | 
      | <h4>Slave Index:</h4>
      | Set the EtherCAT slave index. Following address formats are allowed:
      | <ol>
      | <li> Absolute addressing: a scalar number <<b><tt>n</tt></b>> representing the (zero based) absolute position in the bus.
      | <li> SSId addressing: the Secondary Slave (or 'Alias') Addressing has the form <<b><tt>[alias position]</tt></b>> where <b><tt>alias</tt></b> is the Secondary Slave Id of the EtherCAT slave and <b><tt>position</tt></b> is the offset after the slave with the given <b><tt>alias</tt></b>. The SSId has to be preprogrammed into the slave with other service tools (see 'ethercat alias --help').
      | </ol>
      | 
      | <h4>Device Model:</h4>
      | Choose the device at the Indexed position of the master.
      | 
      | <h4>Channel 1-4 Type:</h4>
      | Choose the output type of the channel.
      | 
      | <h4>DC Mode:</h4>
      | Choose the DC Mode for the module.
      | 
      | <h4>DC Customized:</h4>
      | 
      | <<b><tt>[AssignActivate, CycleTimeSync0, CycleTimeSync0Factor, ShiftTimeSync0, ShiftTimeSync0Factor, ...
      | ShiftTimeSync0Input, CycleTimeSync1, CycleTimeSync1Factor, ShiftTimeSync1, ShiftTimeSync1Factor]</tt></b>>
      | 
      | <ul>
      | <li><<b><tt>AssignActivate:</tt></b>> Value for DC-mode setting
      | <li><<b><tt>CycleTimeSync0:</tt></b>> CycleTimeSync0 Value
      | <li><<b><tt>CycleTimeSync0Factor:</tt></b>> 1 or 0. If CycleTimeSync0Factor equals one the cycletimesync0 value is internally set to the process cycletime.
      | <li><<b><tt>ShiftTimeSync0:</tt></b>> ShiftTimeSync0 Value
      | <li><<b><tt>ShiftTimeSync0Factor:</tt></b>> 1 or 0. If ShiftTimeSync0Factor equals one the Slave is synced on the input event
      | <li><<b><tt>ShiftTimeSync0Input:</tt></b>> 1 or 0. If ShiftTimeSync0Input equals one the Slave is synced on the input event
      | <li><<b><tt>CycleTimeSync1:</tt></b>> CycleTimeSync1 Value
      | <li><<b><tt>CycleTimeSync1Factor:</tt></b>> 1 or 0. If CycleTimeSync1Factor equals one the CycletTimesSync1 value is internally set to the process cycletime.
      | <li><<b><tt>ShiftTimeSync1:</tt></b>>ShiftTimeSync1 Value
      | <li><<b><tt>ShiftTimeSync1Factor:</tt></b>> ShiftTimeSync1Factor Value
      | </ul>
      | 
      | <h4>Input Type:</h4>
      | <ul>
      | <li>Choose <b>Vector Input</b> to have a single input as a vector
      | with a size corresponding to the channel count of the terminal. This mode also allows a control input and a status output port to be displayed.
      | <li>Choose <b>Separate Inputs</b> to have one input for every channel.
      | </ul>
      | 
      | <p>
      | All input signals are multiplied with the factor <b>Input Scale</b>.
      | 
      | <p>
      | Set the <b>Sample Time</b> for the block. <tt>0</tt> is continuous sample time (runs at the model's base rate). Setting <tt>-1</tt> will try to set the time using back propagation.
      mask StyleString: edit,edit,popup(EP4174-0002),popup(-10...+10 V|0...20 mA|4...20 mA|0...10 V),popup(-10...+10 V|0...20 mA|4...20 mA|0...10 V),popup(-10...+10 V|0...20 mA|4...20 mA|0...10 V),popup(-10...+10 V|0...20 mA|4...20 mA|0...10 V),popup(FreeRun/SM-Synchron|DC-Synchron|DC-Customized),edit,checkbox,edit,edit,edit
      mask CallbackString: ||ep41xx('set')|||||ep41xx('set')||ep41xx('set')|||
      mask Display:
      | fprintf('%s\nM:%s Idx:%s', ...
      |     model, masterStr, positionStr)
  EP41xx_1 : S-Function  FunctionName=ec_slave3  Parameters=Address,rv.SlaveConfig,rv.PortConfig,debug,tsample  SFunctionModules='ecrt_support'  EnableBusSupport=off  mask(EP41xx){master=0, index=1, model=EP4174-0002, type_1=0...10 V, type_2=0...10 V, type_3=0...10 V, type_4=0...10 V, vector=on, gain=, tsample=0, debug=0, dc_mode=FreeRun/SM-Synchron, dc_assign_activate=hex2dec('730'), dc_cycle0=0, dc_cycle0_factor=1, dc_shift0=0, dc_shift0_factor=0, dc_shift0_input=off, dc_cycle1=0, dc_cycle1_factor=1, dc_shift1=140000, dc_shift1_factor=0}
      mask prompts: index "Slave Index"; model "Device Model"; type_1 "Channel 1 Type"; type_2 "Channel 2 Type"; type_3 "Channel 3 Type"; type_4 "Channel 4 Type"; vector "Vector Input"; gain "Input Scale (empty for none)"; tsample "Sample Time (-1 for inherited)"; dc_mode "DC Mode"; dc_assign_activate "Assign Activate"; dc_cycle0 "Cycle Time Sync 0"; dc_cycle0_factor "Factor"; dc_shift0 "Shift Time Sync0"; dc_shift0_factor "Factor"; dc_shift0_input "Shift Time0 Input"; dc_cycle1 "Cycle Time Sync1"; dc_cycle1_factor "Factor"; dc_shift1 "Shift Time Sync1"; dc_shift1_factor "Factor"
      mask help: Beckhoff Analog Output Fieldbus Box
      mask init:
      | Address = getEtherCATAddress(gcb, master, index, tsample);
      | 
      | rv = ep41xx_1.configure(model,vector,...
      |     EtherCATSlave.configureScale(2^15,gain),...
      |     [dc_mode, dc_assign_activate, ...
      |      dc_cycle0, dc_cycle0_factor, ...
      |      dc_shift0, dc_shift0_factor, dc_shift0_input, ...
      |      dc_cycle1, dc_cycle1_factor, ...
      |      dc_shift1, dc_shift1_factor], ...
      |      [type_1; type_2; type_3; type_4]);
      mask Help:
      | This block generically implements the EtherCAT 16-Bit Analog Input Terminal for various fieldbus boxes.
      | <p/>
      | The block input is generally a <tt>double</tt> from the range 0..1 for unipolar terminals and -1..1 for bipolar terminals, where 1 is the highest possible output of the terminal.
      | <p/>
      | Exceeding the input range simply saturates the terminal's output.
      | <p/>
      | The following Terminals are supported:
      | <center>
      | <table width="80%">
      | <tr><td>EP4174</td><td>+/-10V, 0..10V,  Voltage Output or 0..20mA, 4..20mA Current Output</td></tr>
      | </table>
      | </center>
      | <p/>
      | Choose and set the following options:
      | <h4>Master:</h4>
      | Set the EtherCAT Master of this terminal.
      | 
      | <h4>Slave Index:</h4>
      | Set the EtherCAT slave index. Following address formats are allowed:
      | <ol>
      | <li> Absolute addressing: a scalar number <<b><tt>n</tt></b>> representing the (zero based) absolute position in the bus.
      | <li> SSId addressing: the Secondary Slave (or 'Alias') Addressing has the form <<b><tt>[alias position]</tt></b>> where <b><tt>alias</tt></b> is the Secondary Slave Id of the EtherCAT slave and <b><tt>position</tt></b> is the offset after the slave with the given <b><tt>alias</tt></b>. The SSId has to be preprogrammed into the slave with other service tools (see 'ethercat alias --help').
      | </ol>
      | 
      | <h4>Device Model:</h4>
      | Choose the device at the Indexed position of the master.
      | 
      | <h4>Channel 1-4 Type:</h4>
      | Choose the output type of the channel.
      | 
      | <h4>DC Mode:</h4>
      | Choose the DC Mode for the module.
      | 
      | <h4>DC Customized:</h4>
      | 
      | <<b><tt>[AssignActivate, CycleTimeSync0, CycleTimeSync0Factor, ShiftTimeSync0, ShiftTimeSync0Factor, ...
      | ShiftTimeSync0Input, CycleTimeSync1, CycleTimeSync1Factor, ShiftTimeSync1, ShiftTimeSync1Factor]</tt></b>>
      | 
      | <ul>
      | <li><<b><tt>AssignActivate:</tt></b>> Value for DC-mode setting
      | <li><<b><tt>CycleTimeSync0:</tt></b>> CycleTimeSync0 Value
      | <li><<b><tt>CycleTimeSync0Factor:</tt></b>> 1 or 0. If CycleTimeSync0Factor equals one the cycletimesync0 value is internally set to the process cycletime.
      | <li><<b><tt>ShiftTimeSync0:</tt></b>> ShiftTimeSync0 Value
      | <li><<b><tt>ShiftTimeSync0Factor:</tt></b>> 1 or 0. If ShiftTimeSync0Factor equals one the Slave is synced on the input event
      | <li><<b><tt>ShiftTimeSync0Input:</tt></b>> 1 or 0. If ShiftTimeSync0Input equals one the Slave is synced on the input event
      | <li><<b><tt>CycleTimeSync1:</tt></b>> CycleTimeSync1 Value
      | <li><<b><tt>CycleTimeSync1Factor:</tt></b>> 1 or 0. If CycleTimeSync1Factor equals one the CycletTimesSync1 value is internally set to the process cycletime.
      | <li><<b><tt>ShiftTimeSync1:</tt></b>>ShiftTimeSync1 Value
      | <li><<b><tt>ShiftTimeSync1Factor:</tt></b>> ShiftTimeSync1Factor Value
      | </ul>
      | 
      | <h4>Input Type:</h4>
      | <ul>
      | <li>Choose <b>Vector Input</b> to have a single input as a vector
      | with a size corresponding to the channel count of the terminal. This mode also allows a control input and a status output port to be displayed.
      | <li>Choose <b>Separate Inputs</b> to have one input for every channel.
      | </ul>
      | 
      | <p>
      | All input signals are multiplied with the factor <b>Input Scale</b>.
      | 
      | <p>
      | Set the <b>Sample Time</b> for the block. <tt>0</tt> is continuous sample time (runs at the model's base rate). Setting <tt>-1</tt> will try to set the time using back propagation.
      mask StyleString: edit,edit,popup(EP4174-0002),popup(-10...+10 V|0...20 mA|4...20 mA|0...10 V),popup(-10...+10 V|0...20 mA|4...20 mA|0...10 V),popup(-10...+10 V|0...20 mA|4...20 mA|0...10 V),popup(-10...+10 V|0...20 mA|4...20 mA|0...10 V),checkbox,edit,edit,edit,popup(FreeRun/SM-Synchron|DC-Synchron|Custom),edit,min,max,min,max,checkbox,min,max,min,max
      mask CallbackString: |||||||||||EtherCATSlaveBlock().updateCustomDCEnable()||||||||||
      mask TabNameString: Main,Main,Main,Main,Main,Main,Main,Main,Main,Main,Main,Distributed Clocks,Distributed Clocks,Distributed Clocks,Distributed Clocks,Distributed Clocks,Distributed Clocks,Distributed Clocks,Distributed Clocks,Distributed Clocks,Distributed Clocks,Distributed Clocks
      mask Display: fprintf('%s\nM:%i Idx:%s', model, master, mat2str(index))
  EP43xx_0 : S-Function  LoadFcn=ep43xx('check');  FunctionName=ec_slave3  Parameters=Address,rv.SlaveConfig,rv.PortConfig,debug,tsample  SFunctionModules='ecrt_support'  EnableBusSupport=off  mask(EP4374){master=0, index=1, model=EP4374-0002, type_1=0...10 V, type_2=0...10 V, type_3=0...10 V, type_4=0...10 V, status=off, vector=on, dcmode=FreeRun/SM-Synchron, dccustom=[hex2dec('700') 0 1 0 0 0 0 1 80000 0], i_scale=[], o_scale=[], o_offset=[], tau=[], force=off, tsample=0, debug=0}
      mask prompts: index "Slave Index"; model "Device Model"; type_1 "Input type Ch1"; type_2 "Input type Ch2"; type_3 "Output type Ch3"; type_4 "Output type Ch4"; status "Status Output"; vector "Vector IO"; dcmode "DC Mode"; dccustom "DC Customer"; i_scale "Input Scale"; o_scale "Output Scale"; o_offset "Output Offset"; tau "LPF Time Constant (sec)"; force "IO Force"; tsample "Sample Time (-1 for inherited)"
      mask help: Beckhoff Analog Input/Output 16-Bit Fieldbus Box
      mask init:
      | masterStr = '';
      | positionStr = '';
      | [Address masterStr positionStr] = ...
      |     getEtherCATAddress(gcb, master, index, tsample);
      | 
      | ep43xx('set');
      | 
      | rv = get_param(gcbh,'UserData');
      | 
      | rowcount = numel(rv.SlaveConfig.sm{1}{3}) ...
      |          + numel(rv.SlaveConfig.sm{2}{3});
      | 
      | rv.SlaveConfig.sdo = num2cell(horzcat(...
      |     hex2dec('F800')*ones(rowcount,1),...
      |     (1:rowcount)',...
      |     16*ones(rowcount,1),...
      |     [type_1; type_2; type_3; type_4] - 1));
      mask Help: web(etherlab_help_path('ep43xx.html'), '-helpbrowser')
      mask StyleString: edit,edit,popup(EP4374-0002),popup(-10...+10 V|0...20 mA|4...20 mA|0...10 V),popup(-10...+10 V|0...20 mA|4...20 mA|0...10 V),popup(-10...+10 V|0...20 mA|4...20 mA|0...10 V),popup(-10...+10 V|0...20 mA|4...20 mA|0...10 V),checkbox,checkbox,popup(FreeRun/SM-Synchron|DC-Synchron|DC-Customized),edit,edit,edit,edit,edit,checkbox,edit,edit
      mask CallbackString: ||ep43xx('set');|||||ep43xx('set');|ep43xx('set');|ep43xx('ui');||||||||
      mask Display:
      | fprintf('%s\nAnalog IO\nM:%s Idx:%s', ...
      |     model, masterStr, positionStr);
  EP43xx_1 : S-Function  FunctionName=ec_slave3  Parameters=Address,rv.SlaveConfig,rv.PortConfig,debug,tsample  SFunctionModules='ecrt_support'  EnableBusSupport=off  mask(EP4374){master=0, index=1, model=EP4374-0002, vector=on, tsample=0, debug=, type_1=0...10 V, type_2=-10...+10 V, filter=Off, status=off, o_gain=, o_offset=, tau=, type_3=-10...+10 V, type_4=-10...+10 V, i_gain=, dc_mode=FreeRun/SM-Synchron, dc_assign_activate=hex2dec('700'), dc_cycle0=0, dc_cycle0_factor=1, dc_shift0=0, dc_shift0_factor=0, dc_shift0_input=off, dc_cycle1=0, dc_cycle1_factor=1, dc_shift1=80000, dc_shift1_factor=0}
      mask prompts: index "Slave Index"; model "Device Model"; vector "Vector IO"; tsample "Sample Time (-1 for inherited)"; type_1 "Analog Input type Ch1"; type_2 "Analog Input type Ch2"; o_gain "Scale"; o_offset "Offset"; tau "LPF Time Constant (sec)"; type_3 "Analog Output type Ch3"; type_4 "Analog Output type Ch4"; i_gain "Scale"; dc_mode "DC Mode"; dc_assign_activate "Assign Activate"; dc_cycle0 "Cycle Time Sync 0"; dc_cycle0_factor "Factor"; dc_shift0 "Shift Time Sync0"; dc_shift0_factor "Factor"; dc_shift0_input "Shift Time0 Input"; dc_cycle1 "Cycle Time Sync1"; dc_cycle1_factor "Factor"; dc_shift1 "Shift Time Sync1"; dc_shift1_factor "Factor"
      mask help: Beckhoff Analog Input/Output 16-Bit Fieldbus Box
      mask init:
      | Address = getEtherCATAddress(gcb, master, index, tsample);
      | 
      | rv = ep43xx_1.configure(model,status,vector,...
      |     EtherCATSlave.configureScale(2^15,o_gain,o_offset,tau),...
      |     EtherCATSlave.configureScale(2^15,i_gain),...
      |     [dc_mode, dc_assign_activate, ...
      |      dc_cycle0, dc_cycle0_factor, ...
      |      dc_shift0, dc_shift0_factor, dc_shift0_input, ...
      |      dc_cycle1, dc_cycle1_factor, ...
      |      dc_shift1, dc_shift1_factor],...
      |      filter,[type_1,type_2,type_3,type_4]);
      mask Help: web(etherlab_help_path('ep43xx.html'), '-helpbrowser')
      mask StyleString: edit,edit,popup(EP4374-0002),checkbox,edit,edit,popup(-10...+10 V|0...20 mA|4...20 mA|0...10 V),popup(-10...+10 V|0...20 mA|4...20 mA|0...10 V),popup(Off|50Hz FIR|60Hz FIR|IIR 1|IIR 2|IIR 3|IIR 4|IIR 5|IIR 6|IIR 7|IIR 8),checkbox,edit,edit,edit,popup(-10...+10 V|0...20 mA|4...20 mA|0...10 V),popup(-10...+10 V|0...20 mA|4...20 mA|0...10 V),edit,popup(FreeRun/SM-Synchron|DC-Synchron|Custom),edit,min,max,min,max,checkbox,min,max,min,max
      mask CallbackString: ||||||||||||||||EtherCATSlaveBlock().updateCustomDCEnable()||||||||||
      mask TabNameString: Main,Main,Main,Main,Main,Main,Input,Input,Input,Input,Input,Input,Input,Output,Output,Output,Distributed Clocks,Distributed Clocks,Distributed Clocks,Distributed Clocks,Distributed Clocks,Distributed Clocks,Distributed Clocks,Distributed Clocks,Distributed Clocks,Distributed Clocks,Distributed Clocks
      mask Display: fprintf('%s\nAnalog IO\nM:%iIdx:%s', model, master, mat2str(index));
  Infrastructure : S-Function  FunctionName=ec_slave3  Parameters=Address,rv.SlaveConfig,rv.PortConfig,debug,tsample  SFunctionModules='ecrt_support'  EnableBusSupport=off  mask(EKxxxx){master=0, index=1, model=EK1100, vector=off, tsample=0, debug=0}
      mask prompts: index "Slave Index"; model "Device Model"; vector "Vector output"; tsample "Sample Time / Domain"
      mask help:
      | EtherCAT Infrastructure Slaves.
      |
      | Including these slaves (even if they don't have I/Os)
      | will create slave configurations, which will cause them to go into the
      | operational state.
      mask init:
      | Address = getEtherCATAddress(gcb, master, index, tsample);
      | 
      | rv = ekxxxx().configure(model,vector);
      |  
      | EtherCATSlaveBlock().setPortNames(...
      |     {rv.PortConfig.input.portname}, ...
      |     {rv.PortConfig.output.portname},model);
      settings: AttributesFormatString=%<model>\nM:%<master> Id:%<index>
      mask Help: web(etherlab_help_path('ekxxxx.html'), '-helpbrowser')
      mask StyleString: edit,edit,popup(EK1100|EK1100-0030|EK1101|EK1101-0080|EK1110|EK1122|EK1122-0080|EK1200|EK1501|EK1501-0010|EK1521|EK1521-0010|EK1541|EK1561|EK1814|EK1818|EK1828|EK1828-0010|CX1100-0004),checkbox,edit,edit
      mask Display: disp('EK1100')
